simulink model "OcularMotorLabModel_2023_08_25_M22b"  (R2023a)
settings: Solver=FixedStepAuto  StartTime=tStart  StopTime=tFinal  FixedStep=0.001  RelTol=1e-3
undefined symbols (not defined in the file or in its folder): Asp, Asp1, Asp2, e0sp, gaussian, Gpc, GPos, Gsl, psi, Psp1, RotFbk, SatSp, sigbuilder_block, SomFbk, T1, T2, Tccanal, Tcn, Tcr, Tcsp, TCvs, tdm, tdsp1, tdsp2, tdsp3, tdv, Tsl, Tz, w
libraries: matrix_library x10, vrlib x8, simulink_extras x5, simulink x1
(part 1 of 2)
settings Model: Creator=raulr  LastModifiedBy=jom
settings DebuggingCC: UnconnectedInputMsg=warning  UnconnectedOutputMsg=warning  UnconnectedLineMsg=warning
settings ModelReferenceCC: EnableRefExpFcnMdlSchedulingChecks=on
settings RTWCC: DLArmComputeVersion=19.05

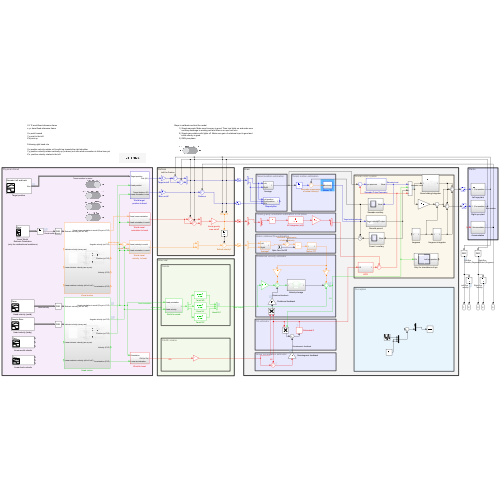
[thumbnail: Simulink's stored preview of the top-level diagram]
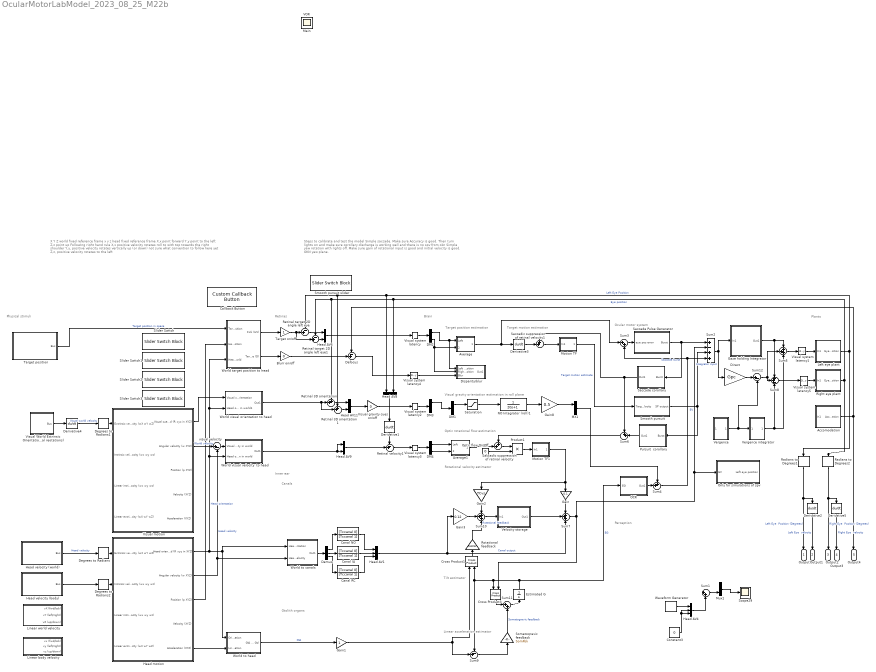
== system OcularMotorLabModel_2023_08_25_M22b ==
  note: Plants
  note: Steps to calibrate and test the model
      | Simple saccade. Make sure Accuracy is good. Then turn lights on and make sure corollary discharge is working well and there is no spv from okn
      | Simple yaw rotation with lights off. Make sure gain of rotational input is good and initial velocity is good.
      | OKN yaw plane.
  note: X Y Z world fixed reference frame
      | x y z head fixed reference frame
      |
      | X,x point forward
      | Y,y point to the left
      | Z,z point up
      |
      | Following right hand rule
      |
      | X,x positive velocity rotates roll to with top towards the right shoulder
      | Y,y, positive velocity rotates vertically up (or down) not sure what convention to follow here yet
      | Z,z, positive velocity rotates to the left
  note: Brain
  note: Ocular motor system
  note: Perception
  note: Optic rotational flow estimation
  note: Rotational velocity estimator
  note: Linear acceleration estimator
  note: Tilt estimator
  note: Retinas
  note: Otolith organs
  note: Canals
  note: Inner ear
  note: Physical stimuli
  note: Visual gravity orientation estimation in roll plane
  note: Target motion estimation
  note: Target position estimation
  Accomodation : Subsystem
  Average : Subsystem
  Average1 : Subsystem
  Blurr on/off : Gain  Gain=0
  Callback Button : CustomCallbackButton  Configuration="{\"components\":[{\"name\":\"BackgroundImageComponent\",\"settings\":{\"image\":{\"size\":[0,0],\"src\":\"default\",\"srcOrientation\":\"Right\"},\"position\":[0,0,1,1]}},{\"name\":\"ButtonStateComponent\",\"settings\":{\"buttonType\":\"momentary\",\"clickFcn\":\"%% Set parameters\\ntStart = 0;\\ntFinal = 60;\\n\\n\\n%% General\\ntdv = 0.050; % visual latency\\ntdm = 0.030; % Motor latency\\n\\n\\n%% plant\\nTz = 0.08;\\nT1 = 0.3;\\nT2 = 0.01; % 0.012\\nw = 200;\\npsi = 1.2;\\n\\n\\n%% Saccade system\\nGpc = 0.06;     % Gain of conjugate pulse\\nGsl = 0.165;    % Gain of slide\\nTsl = Tz;     % Tc slide\\nTcn = 20;       % Tc conjugate neural integrator\\nTcr = Tcn;       % Tc conjugate resettable integrator\\n\\nTep = 0.003;    % Tc motor error pole\\nDelC = 0.006;   % Saccade local feedback delay\\ne0 = 5;         \\nAL = 440;\\nAR = 440;\\nlL = 10;\\nLR = 10;\\n\\n%% Smooth pursuit\\ntdsp1 = 0.015;\\ntdsp2 = 0.035;\\ntdsp3 = 0.030;\\n\\nTcsp = 0.007;\\ne0sp = 4;\\nAsp1 = 10;\\nAsp2 = 5;\\nAsp = 1.1;\\nPsp1 = 0.95;\\nTcsp2 = 0.015;\\nSatSp = 90;\\n\\n%% Vestibular system\\nTccanal = 5;\\nTCvs = 11.5;\\nRotFbk = 0.38;\\nSomFbk = 0.65;\\n\\n%% Integrator\\nGPos = 0.02;\",\"onValue\":1,\"position\":[0,0,1,1],\"pressDelay\":\"500\",\"pressFcn\":\"\",\"repeatInterval\":\"0\",\"states\":[{\"horizontalAlignment\":\"center\",\"image\":{\"position\":[0,0,1,1],\"size\":[1,1],\"src\":\"default\",\"srcOrientation\":\"Right\"},\"label\":{\"color\":[0.01176470588,0.01176470588,0.01176470588,1],\"icon\":{\"size\":[0,0],\"src\":\"default\",\"srcOrientation\":\"Right\"},\"iconPlacement\":\"left\",\"opacity\":1,\"show\":true,\"text\":{\"content\":\"Click to initialize\",\"font\":\"Helvetica\",\"fontSize\":13.865820000000001}},\"labelOffset\":[0,0],\"verticalAlignment\":\"middle\"},{\"horizontalAlignment\":\"center\",\"image\":{\"position\":[0,0,1,1],\"size\":[1,1],\"src\":\"default\",\"srcOrientation\":\"Right\"},\"label\":{\"color\":[0.01176470588,0.01176470588,0.01176470588,1],\"icon\":{\"size\":[0,0],\"src\":\"default\",\"srcOrientation\":\"Right\"},\"iconPlacement\":\"left\",\"opacity\":1,\"show\":true,\"text\":{\"content\":\"Click to initialize\",\"font\":\"Helvetica\",\"fontSize\":13.865820000000001}},\"labelOffset\":[0,0],\"verticalAlignment\":\"middle\"},{\"horizontalAlignment\":\"center\",\"image\":{\"position\":[0,0,1,1],\"size\":[1,1],\"src\":\"default\",\"srcOrientation\":\"Right\"},\"label\":{\"color\":[0.01176470588,0.01176470588,0.01176470588,1],\"icon\":{\"size\":[0,0],\"src\":\"default\",\"srcOrientation\":\"Right\"},\"iconPlacement\":\"left\",\"opacity\":1,\"show\":true,\"text\":{\"content\":\"Click to initialize\",\"font\":\"Helvetica\",\"fontSize\":13.865820000000001}},\"labelOffset\":[0,0],\"verticalAlignment\":\"middle\"},{\"horizontalAlignment\":\"center\",\"image\":{\"position\":[0,0,1,1],\"size\":[1,1],\"src\":\"default\",\"srcOrientation\":\"Right\"},\"label\":{\"color\":[0.01176470588,0.01176470588,0.01176470588,1],\"icon\":{\"size\":[0,0],\"src\":\"default\",\"srcOrientation\":\"Right\"},\"iconPlacement\":\"left\",\"opacity\":1,\"show\":true,\"text\":{\"content\":\"Click to initialize\",\"font\":\"Helvetica\",\"fontSize\":13.865820000000001}},\"labelOffset\":[0,0],\"verticalAlignment\":\"middle\"}]}},{\"name\":\"ForegroundImageComponent\",\"settings\":{\"image\":{\"size\":[0,0],\"src\":\"default\",\"srcOrientation\":\"Right\"},\"isForeground\":1,\"position\":[0,0,1,1]}}],\"settings\":{\"BindingType\":\"standalone\",\"backgroundColor\":[244,244,244,1],\"backgroundOffset\":0.2,\"backgroundOpacity\":1,\"fixedAspectRatio\":\"off\",\"foregroundColor\":[0.01176470588,0.01176470588,0.01176470588,1],\"migratedFromLegacy\":true,\"useBackgroundColor\":true,\"variant\":\"callback\",\"version\":\"R2023a\"},\"type\":\"Button\"}"  CustomBackgroundColor="{\"color\":[0.9568627451,0.9568627451,0.9568627451],\"show\":true}"
  Canal IA : TransferFcn  Numerator=[Tccanal 0]  Denominator=[Tccanal 1]
  Canal NO : TransferFcn  Numerator=[Tccanal 0]  Denominator=[Tccanal 1]
  Canal RC : TransferFcn  Numerator=[Tccanal 0]  Denominator=[Tccanal 1]
  Constant3 : Constant  Value=0
  Cross Product1 : vrlib/Utilities/Cross Product
  Cross Product3 : vrlib/Utilities/Cross Product
  DM1 : Demux  Outputs=3
  DM2 : Demux  Outputs=2
  DM3 : Demux  Outputs=2
  DM4 : Demux  Outputs=2
  Defocus : Sum  Inputs=-+|
  Degrees to Radians : simulink_extras/Transformations/Degrees to Radians
  Degrees to Radians1 : simulink_extras/Transformations/Degrees to Radians
  Degrees to Radians2 : simulink_extras/Transformations/Degrees to Radians
  Demux : Demux  Outputs=3
  Derivative{1..5} (5 alike) : Derivative
  Direct : Gain  Gain=Gpc
  Disparity/blur : Subsystem
  Estimated G : Integrator  InitialCondition=[0 0 -1]'
  Gain : Gain  Gain=0.1
  Gain1 : Gain
  Gain2 : Gain  Gain=TCvs
  Gain3 : Gain  Gain=0.12
  Gain8 : Gain  Gain=0.5
  Gaze holding Integrator : Subsystem
  Head AV1 : Mux  Inputs=3
  Head AV{6,8..9,11} (4 alike) : Mux  Inputs=2
  Head AV4 : Mux  Inputs=3
  Head motion : Subsystem
  Head velocity (body) : Subsystem  Tag=STV Subsys  LoadFcn=sigbuilder_block('load');  StartFcn=sigbuilder_block('start');  StopFcn=sigbuilder_block('stop');  ClipboardFcn=sigbuilder_block('clipboard');  mask(Sigbuilder block){tuvar=[0:10]}
      mask help: Simulink:masks:SigbuilderBlock_MD
      mask init:
      | if ~strcmp(get_param(bdroot(gcbh),'SimulationStatus'),'stopped') tuvar = sigbuilder_block('maskInit'); end
      settings: CopyFcn=sigbuilder_block('copy');  DeleteFcn=sigbuilder_block('delete');  ModelCloseFcn=sigbuilder_block('modelClose');  PreSaveFcn=sigbuilder_block('preSave');  PauseFcn=sigbuilder_block('pause');  ContinueFcn=sigbuilder_block('continue');  NameChangeFcn=sigbuilder_block('namechange');  OpenFcn=sigbuilder_block('open',[5.4 5.4 1141.2 580.8 ]);  CloseFcn=sigbuilder_block('close');
      mask Display: plot(0, 0, 100, 100,[2, 2, 32, 32, 2], [68, 8, 8, 68, 68],[32, 2], [38, 38], [32, 19, 2],[53, 60, 44], [32, 17, 17, 2],[16, 16, 31, 31]);txt = getActiveGroup(gcbh);text(2, 100, txt,'verticalAlignment', 'top');
  Head velocity (world) : Subsystem  Tag=STV Subsys  LoadFcn=sigbuilder_block('load');  StartFcn=sigbuilder_block('start');  StopFcn=sigbuilder_block('stop');  ClipboardFcn=sigbuilder_block('clipboard');  mask(Sigbuilder block){tuvar=[0:10]}
      mask help: Simulink:masks:SigbuilderBlock_MD
      mask init:
      | if ~strcmp(get_param(bdroot(gcbh),'SimulationStatus'),'stopped') tuvar = sigbuilder_block('maskInit'); end
      settings: CopyFcn=sigbuilder_block('copy');  DeleteFcn=sigbuilder_block('delete');  ModelCloseFcn=sigbuilder_block('modelClose');  PreSaveFcn=sigbuilder_block('preSave');  PauseFcn=sigbuilder_block('pause');  ContinueFcn=sigbuilder_block('continue');  NameChangeFcn=sigbuilder_block('namechange');  OpenFcn=sigbuilder_block('open',[2616 248.4 1141.2 580.8 ]);  CloseFcn=sigbuilder_block('close');
      mask Display: plot(0, 0, 100, 100,[2, 2, 32, 32, 2], [68, 8, 8, 68, 68],[32, 2], [38, 38], [32, 19, 2],[53, 60, 44], [32, 17, 17, 2],[16, 16, 31, 31]);txt = getActiveGroup(gcbh);text(2, 100, txt,'verticalAlignment', 'top');
  Left eye plant : Subsystem
  Linear body velocity : Subsystem  Tag=STV Subsys  LoadFcn=sigbuilder_block('load');  StartFcn=sigbuilder_block('start');  StopFcn=sigbuilder_block('stop');  ClipboardFcn=sigbuilder_block('clipboard');  mask(Sigbuilder block){tuvar=[0:10]}
      mask help: Simulink:masks:SigbuilderBlock_MD
      mask init:
      | if ~strcmp(get_param(bdroot(gcbh),'SimulationStatus'),'stopped') tuvar = sigbuilder_block('maskInit'); end
      settings: CopyFcn=sigbuilder_block('copy');  DeleteFcn=sigbuilder_block('delete');  ModelCloseFcn=sigbuilder_block('modelClose');  PreSaveFcn=sigbuilder_block('preSave');  PauseFcn=sigbuilder_block('pause');  ContinueFcn=sigbuilder_block('continue');  NameChangeFcn=sigbuilder_block('namechange');  OpenFcn=sigbuilder_block('open',[352.5 317 1141 398 ]);  CloseFcn=sigbuilder_block('close');
      mask Display: plot(0, 0, 100, 100,[2, 2, 32, 32, 2], [68, 8, 8, 68, 68],[32, 2], [38, 38], [32, 19, 2],[53, 60, 44], [32, 17, 17, 2],[16, 16, 31, 31]);txt = getActiveGroup(gcbh);text(2, 100, txt,'verticalAlignment', 'top');
  Linear world velocity : Subsystem  Tag=STV Subsys  LoadFcn=sigbuilder_block('load');  StartFcn=sigbuilder_block('start');  StopFcn=sigbuilder_block('stop');  ClipboardFcn=sigbuilder_block('clipboard');  mask(Sigbuilder block){tuvar=[0:10]}
      mask help: Simulink:masks:SigbuilderBlock_MD
      mask init:
      | if ~strcmp(get_param(bdroot(gcbh),'SimulationStatus'),'stopped') tuvar = sigbuilder_block('maskInit'); end
      settings: CopyFcn=sigbuilder_block('copy');  DeleteFcn=sigbuilder_block('delete');  ModelCloseFcn=sigbuilder_block('modelClose');  PreSaveFcn=sigbuilder_block('preSave');  PauseFcn=sigbuilder_block('pause');  ContinueFcn=sigbuilder_block('continue');  NameChangeFcn=sigbuilder_block('namechange');  OpenFcn=sigbuilder_block('open',[448.5 188.5 1141 397.7 ]);  CloseFcn=sigbuilder_block('close');
      mask Display: plot(0, 0, 100, 100,[2, 2, 32, 32, 2], [68, 8, 8, 68, 68],[32, 2], [38, 38], [32, 19, 2],[53, 60, 44], [32, 17, 17, 2],[16, 16, 31, 31]);txt = getActiveGroup(gcbh);text(2, 100, txt,'verticalAlignment', 'top');
  MX1 : Mux  Inputs=3
  Motion TF : Subsystem
  Motion TF1 : Subsystem
  Mux1 : Mux  Inputs=2
  NO Integrator (roll)1 : TransferFcn  Denominator=[20 1]
  OCR : Subsystem
  Only for simulations of spv : Subsystem
  Optic flow On/Off : Constant  Value=0
  Product1 : Product
  Pursuit  corollary : Subsystem
  Radians to Degrees1 : simulink_extras/Transformations/Radians to Degrees
  Radians to Degrees2 : simulink_extras/Transformations/Radians to Degrees
  Retinal 3D orientation : Sum  Inputs=++|
  Retinal 3D orientation1 : Sum  Inputs=++|
  Retinal target 2D angle left eye : Sum  Inputs=-+|
  Retinal target 2D angle left eye1 : Sum  Inputs=-+|
  Retinal velocity1 : Sum  Inputs=-+|
  Right eye plant : Subsystem
  Rotational feedback : Gain  Gain=RotFbk
  Saccade Pulse Generator : Subsystem
  Saccade corollary : Subsystem
  Saccadic suppression of retinal velocity : Sum  Inputs=++|
  Saccadic suppression of retinal velocity1 : Sum  Inputs=++|
  Saturation : Saturate  UpperLimit=5*pi/180  LowerLimit=-5*pi/180
  Scope29 : Scope
  Slider Switch{,1..3} (4 alike) : SliderSwitchBlock
      settings: Values={{'Off', 'On'}, [0 1]}
  Smooth pursuit : Subsystem
  Smooth pursuit slider : SliderSwitchBlock
      settings: Values={{'Off', 'On'}, [0 1]}
  Somatogravic feedback : Gain  Gain=SomFbk
  Sum1 : Sum  Inputs=|++
  Sum10 : Sum  Inputs=+++
  Sum11 : Sum  Inputs=|++
  Sum12 : Sum  Inputs=|+-
  Sum2 : Sum  Inputs=+-++
  Sum3 : Sum  Inputs=|++
  Sum4 : Sum  Inputs=++|
  Sum5 : Sum  Inputs=+++
  Sum6 : Sum  Inputs=++|
  Sum7 : Sum  Inputs=+++
  Sum8 : Sum  Inputs=++-
  Sum9 : Sum  Inputs=-+|
  Target on/off : Gain
  Target position : Subsystem  Tag=STV Subsys  LoadFcn=sigbuilder_block('load');  StartFcn=sigbuilder_block('start');  StopFcn=sigbuilder_block('stop');  ClipboardFcn=sigbuilder_block('clipboard');  mask(Sigbuilder block){tuvar=[0:10]}
      mask help: Simulink:masks:SigbuilderBlock_MD
      mask init:
      | if ~strcmp(get_param(bdroot(gcbh),'SimulationStatus'),'stopped') tuvar = sigbuilder_block('maskInit'); end
      settings: CopyFcn=sigbuilder_block('copy');  DeleteFcn=sigbuilder_block('delete');  ModelCloseFcn=sigbuilder_block('modelClose');  PreSaveFcn=sigbuilder_block('preSave');  PauseFcn=sigbuilder_block('pause');  ContinueFcn=sigbuilder_block('continue');  NameChangeFcn=sigbuilder_block('namechange');  OpenFcn=sigbuilder_block('open',[2766.6 334.8 1141.2 502.8 ]);  CloseFcn=sigbuilder_block('close');
      mask Display: plot(0, 0, 100, 100,[2, 2, 32, 32, 2], [68, 8, 8, 68, 68],[32, 2], [38, 38], [32, 19, 2],[53, 60, 44], [32, 17, 17, 2],[16, 16, 31, 31]);txt = getActiveGroup(gcbh);text(2, 100, txt,'verticalAlignment', 'top');
  Velocity storage : Subsystem
  Vergence : Subsystem
  Vergence integrator : Subsystem
  Visual World Extrinsic Orientation (only for unidirectional reotations) : Subsystem  Tag=STV Subsys  LoadFcn=sigbuilder_block('load');  StartFcn=sigbuilder_block('start');  StopFcn=sigbuilder_block('stop');  ClipboardFcn=sigbuilder_block('clipboard');  mask(Sigbuilder block){tuvar=[0:10]}
      mask help: Simulink:masks:SigbuilderBlock_MD
      mask init:
      | if ~strcmp(get_param(bdroot(gcbh),'SimulationStatus'),'stopped') tuvar = sigbuilder_block('maskInit'); end
      settings: CopyFcn=sigbuilder_block('copy');  DeleteFcn=sigbuilder_block('delete');  ModelCloseFcn=sigbuilder_block('modelClose');  PreSaveFcn=sigbuilder_block('preSave');  PauseFcn=sigbuilder_block('pause');  ContinueFcn=sigbuilder_block('continue');  NameChangeFcn=sigbuilder_block('namechange');  OpenFcn=sigbuilder_block('open',[389.4 19.2 1909.2 907.8 ]);  CloseFcn=sigbuilder_block('close');
      mask Display: plot(0, 0, 100, 100,[2, 2, 32, 32, 2], [68, 8, 8, 68, 68],[32, 2], [38, 38], [32, 19, 2],[53, 60, 44], [32, 17, 17, 2],[16, 16, 31, 31]);txt = getActiveGroup(gcbh);text(2, 100, txt,'verticalAlignment', 'top');
  Visual gravity cues on/off : Gain  Gain=0
  Visual motion : Subsystem
  Visual system latency{,2..4} (4 alike) : TransportDelay  DelayTime=tdv
  Visual system latency1 : TransportDelay  DelayTime=tdm
  Visual system latency5 : TransportDelay  DelayTime=tdm
  Waveform Generator : simulink/Sources/Waveform Generator  OutMin=[]  OutMax=[]  OutDataTypeStr=double  SelectedSignal=1  Signals=gaussian(0,0.1,1)  BlockNames=MultiportSwitch_125da93d47db44d  SampleTime=0.1
  World target position to head : Subsystem
  World to canals : Subsystem
  World to head : Subsystem
  World visual orientation to head : Subsystem
  World visual velocity  to head : Subsystem
  visual velocity : Sum  Inputs=|+-
  Output : Outport
  Output1 : Outport  Port=2
  Output2 : Outport  Port=3
  Output3 : Outport  Port=4
  Output4 : Outport  Port=5
  Main : Scope
  VOR : Scope
  wires:
  Sum7/1 -> Only for simulations of spv/1(EV), Sum2/2, Cross Product3/2  "EV"
  Sum9/1 -> Somatogravic feedback/1
  Cross Product3/1 -> Sum11/1
  Estimated G/1 -> Cross Product3/1, Sum9/1, Cross Product1/2, OCR/1(EG)  "EG"
  Cross Product1/1 -> Rotational feedback/1
  Demux/1 -> Canal NO/1
  Demux/2 -> Canal IA/1
  Canal IA/1 -> Head AV1/2
  Canal NO/1 -> Head AV1/1
  Canal RC/1 -> Head AV1/3
  Demux/3 -> Canal RC/1
  Head AV1/1 -> Gain3/1, Sum7/3  "Canal output"
  Head velocity (world)/1(Bus) -> Degrees to Radians/1  "Head velocity"
  Sum11/1 -> Estimated G/1
  Rotational feedback/1 -> Sum10/3  "Rotational feedback"
  Somatogravic feedback/1 -> Sum11/2  "Somatogravic feedback"
  Gaze holding Integrator/1(Out1) -> Sum5/1, Sum8/1
  Gain1/1 -> Cross Product1/1, Sum9/2
  Gain3/1 -> Sum10/2
  Motion TF1/1(Out1) -> Gain/1, Gain2/1
  Gain/1 -> Sum7/1
  Radians to Degrees1/1 -> Derivative2/1, Output/1  "Left Eye  Position (Degrees)"
  NO Integrator (roll)1/1 -> Gain8/1
  MX1/1 -> Sum4/1
  Derivative4/1 -> Degrees to Radians1/1  "Visual world velocity"
  Sum1/1 -> Mux1/2
  Mux1/1 -> Scope29/1
  Constant3/1 -> Head AV4/2, Head AV4/3
  Waveform Generator/1 -> Head AV4/1
  Head AV4/1 -> Sum1/2
  Saccade Pulse Generator/1(Burst) -> Saccade corollary/1(Burst), Sum2/1  "Saccade burst"
  Sum2/1 -> Direct/1, Gaze holding Integrator/1(In1)  "Integrator input"
  Product1/1 -> Motion TF1/1(In1)
  Saccadic suppression of retinal velocity/1 -> Product1/1
  Sum4/1 -> Sum3/2, Sum2/4
  Head velocity (body)/1(Bus) -> Degrees to Radians2/1
  Degrees to Radians2/1 -> Head motion/2(Intrinsic velocity (wx wy wz))
  Degrees to Radians/1 -> Head motion/1(Extrinsic velocity (wX wY wZ))
  Head motion/1(Head orientation in world (R xyz in XYZ)) -> World to canals/1(Head orientation), World to head/1(Orientation), World visual velocity  to head/2(Head orientation in world), World target position to head/3(Head orientation in world), World visual orientation to head/2(Head orientation in world1)  "Head orientation"
  Head motion/5(Acceleration (XYZ)) -> World to head/2(Linear acceleration)
  Head motion/2(Angular velocity (w XYZ)) -> visual velocity/2, World to canals/2(Head velocity)  "Head velocity"
  Degrees to Radians1/1 -> Visual motion/1(Extrinsic velocity (wX wY wZ))
  visual velocity/1 -> World visual velocity  to head/1(Visual velocity in world)
  Target position/1(Bus) -> World target position to head/1(Target position)  "Target position in space"
  Head motion/3(Position (p XYZ)) -> World target position to head/2(Head position)
  Visual motion/1(Visual cues orientation in world (R xyz in XYZ)) -> World visual orientation to head/1(Visual cues orientation)
  Visual motion/2(Angular velocity (w XYZ)) -> visual velocity/1  "World velocity"
  World visual velocity  to head/1(Out1) -> Head AV9/2, Head AV9/1
  World to canals/1(Out1) -> Demux/1
  World target position to head/1(Fick (HV)) -> Target on/off/1
  World to head/1(GIA (in Gs)) -> Gain1/1  "GIA"
  Sum3/1 -> Saccade Pulse Generator/1(eye pos error)
  OCR/1(Out1) -> Sum4/2
  Saturation/1 -> NO Integrator (roll)1/1
  Optic flow On/Off/1 -> Product1/2
  DM1/1 -> Saturation/1
  Gain8/1 -> MX1/1
  Average/1(Out1) -> Sum3/1, Derivative3/1
  Motion TF/1(Target velocity) -> Smooth pursuit/1(Target velocity)  "Target motion estimate"
  DM2/1 -> Disparity/blur/1(Left position), Average/1(Left)
  DM3/1 -> DM1/1
  Retinal velocity1/1 -> Visual system latency3/1
  Gain2/1 -> Sum10/1
  Derivative1/1 -> Retinal velocity1/1
  Visual system latency3/1 -> DM4/1
  Saccade corollary/1(Out1) -> Saccadic suppression of retinal velocity1/1, Sum6/1
  Smooth pursuit/1(SP output) -> Sum2/3, Pursuit  corollary/1(Burst)
  World target position to head/2(Target distance (D)) -> Blurr on/off/1
  Defocus/1 -> Visual system latency4/1
  Head AV6/1 -> Visual system latency/1
  DM2/2 -> Average/2(Right), Disparity/blur/2(Right position)
  Visual system latency4/1 -> Disparity/blur/3(Blur)
  Average1/1(Out1) -> Saccadic suppression of retinal velocity/2
  DM4/2 -> Average1/2(Right)
  Visual system latency/1 -> DM2/1
  Visual system latency2/1 -> DM3/1
  Head AV8/1 -> Derivative1/1
  DM4/1 -> Average1/1(Left)
  Head AV9/1 -> Retinal velocity1/2
  Target on/off/1 -> Retinal target 2D angle left eye1/2, Retinal target 2D angle left eye/2
  World visual orientation to head/1(Out1) -> Retinal 3D orientation/2, Retinal 3D orientation1/2
  Retinal target 2D angle left eye/1 -> Head AV6/1
  Retinal target 2D angle left eye1/1 -> Head AV6/2
  Derivative3/1 -> Saccadic suppression of retinal velocity1/2
  Saccadic suppression of retinal velocity1/1 -> Motion TF/1(In1)
  Sum6/1 -> Saccadic suppression of retinal velocity/1
  Pursuit  corollary/1(Out1) -> Sum6/2
  Right eye plant/1(Eye position) -> Radians to Degrees2/1, Head AV8/2, Retinal 3D orientation/1, Retinal target 2D angle left eye1/1  "Eye position"
  Sum8/1 -> Visual system latency5/1
  Accomodation/1(Accomodation) -> Output4/1, Defocus/1
  ? -> Accomodation/1(In1)
  Sum5/1 -> Visual system latency1/1
  Left eye plant/1(Eye position) -> Radians to Degrees1/1, Retinal target 2D angle left eye/1, Retinal 3D orientation1/1, Head AV8/1  "Left Eye Position"
  Blurr on/off/1 -> Defocus/2
  Retinal 3D orientation1/1 -> Head AV11/2
  Retinal 3D orientation/1 -> Head AV11/1
  Head AV11/1 -> Visual gravity cues on/off/1
  Vergence/1(Out1) -> Vergence integrator/1(In1), Sum12/2
  Sum12/1 -> Sum8/2, Sum5/2
  Direct/1 -> Sum12/1
  Vergence integrator/1(Out1) -> Sum8/3, Sum5/3
  Visual system latency1/1 -> Left eye plant/1(In1)
  Visual system latency5/1 -> Right eye plant/1(In1)
  Sum10/1 -> Velocity storage/1(In1)
  Velocity storage/1(Out1) -> Sum7/2
  Visual gravity cues on/off/1 -> Visual system latency2/1
  Derivative2/1 -> Output1/1  "Left Eye  velocity"
  Derivative5/1 -> Output3/1  "Right Eye  velocity"
  Radians to Degrees2/1 -> Derivative5/1, Output2/1  "Right Eye  Position (Degrees)"
  Visual World Extrinsic Orientation (only for unidirectional reotations)/1(Bus) -> Derivative4/1

== system OcularMotorLabModel_2023_08_25_M22b/Accomodation ==
  In1 : Inport
  Accomodation : Outport

== system OcularMotorLabModel_2023_08_25_M22b/Average ==
  Left : Inport
  Right : Inport  Port=2
  Constant : Constant  Value=2
  Divide : Product  Inputs=*/
  Sum : Sum  Inputs=|++
  Out1 : Outport
  wires:
  Divide/1 -> Out1/1
  Sum/1 -> Divide/1
  Left/1 -> Sum/1
  Constant/1 -> Divide/2
  Right/1 -> Sum/2

== system OcularMotorLabModel_2023_08_25_M22b/Average1 ==
  Left : Inport
  Right : Inport  Port=2
  Constant : Constant  Value=2
  Divide : Product  Inputs=*/
  Sum : Sum  Inputs=|++
  Out1 : Outport
  wires:
  Divide/1 -> Out1/1
  Sum/1 -> Divide/1
  Left/1 -> Sum/1
  Constant/1 -> Divide/2
  Right/1 -> Sum/2

== system OcularMotorLabModel_2023_08_25_M22b/Disparity//blur ==
  Left position : Inport
  Right position : Inport  Port=2
  Blur : Inport  Port=3
  Out1 : Outport

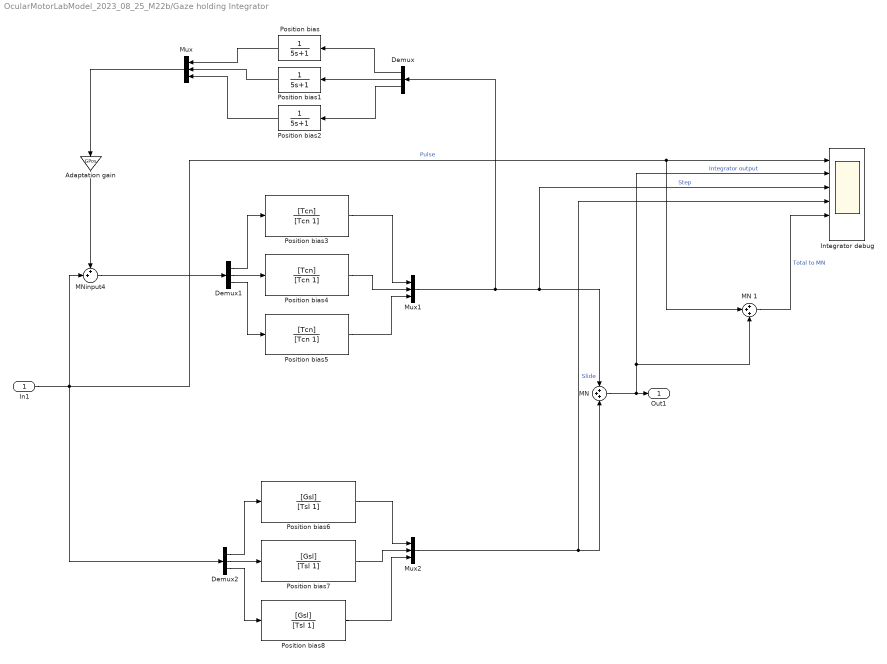
== system OcularMotorLabModel_2023_08_25_M22b/Gaze holding Integrator ==
  In1 : Inport
  Adaptation gain : Gain  Gain=GPos
  Demux : Demux  Outputs=3
  Demux1 : Demux  Outputs=3
  Demux2 : Demux  Outputs=3
  Integrator debug : Scope  NumInputPorts=6
  "MN " : Sum  Inputs=+++  InputSameDT=on  SaturateOnIntegerOverflow=on  OutDataTypeStr=Inherit: Same as first input
  MN 1 : Sum  Inputs=+++  InputSameDT=on  SaturateOnIntegerOverflow=on  OutDataTypeStr=Inherit: Same as first input
  MNinput4 : Sum  Inputs=++|  InputSameDT=on  SaturateOnIntegerOverflow=on  OutDataTypeStr=Inherit: Same as first input
  Mux : Mux  Inputs=3
  Mux1 : Mux  Inputs=3
  Mux2 : Mux  Inputs=3
  Position bias : TransferFcn  Numerator=1  Denominator=[5 1]
  Position bias1 : TransferFcn  Numerator=1  Denominator=[5 1]
  Position bias2 : TransferFcn  Numerator=1  Denominator=[5 1]
  Position bias3 : TransferFcn  Numerator=[Tcn]  Denominator=[Tcn 1]
  Position bias4 : TransferFcn  Numerator=[Tcn]  Denominator=[Tcn 1]
  Position bias5 : TransferFcn  Numerator=[Tcn]  Denominator=[Tcn 1]
  Position bias6 : TransferFcn  Numerator=[Gsl]  Denominator=[Tsl 1]
  Position bias7 : TransferFcn  Numerator=[Gsl]  Denominator=[Tsl 1]
  Position bias8 : TransferFcn  Numerator=[Gsl]  Denominator=[Tsl 1]
  Out1 : Outport
  wires:
  Mux/1 -> Adaptation gain/1
  Demux/1 -> Position bias/1
  Demux/2 -> Position bias1/1
  Demux/3 -> Position bias2/1
  Position bias1/1 -> Mux/2
  Position bias/1 -> Mux/1
  Position bias2/1 -> Mux/3
  MNinput4/1 -> Demux1/1
  Position bias4/1 -> Mux1/2
  Demux1/3 -> Position bias5/1
  Mux1/1 -> Demux/1, Integrator debug/3, "MN "/1  "Step"
  Position bias5/1 -> Mux1/3
  Position bias3/1 -> Mux1/1
  Demux1/2 -> Position bias4/1
  Demux1/1 -> Position bias3/1
  Position bias7/1 -> Mux2/2
  In1/1 -> MN 1/2, Integrator debug/1, MNinput4/2, Demux2/1  "Pulse"
  Demux2/1 -> Position bias6/1
  Position bias6/1 -> Mux2/1
  Demux2/3 -> Position bias8/1
  Position bias8/1 -> Mux2/3
  Demux2/2 -> Position bias7/1
  Mux2/1 -> "MN "/3, Integrator debug/4  "Slide"
  "MN "/1 -> MN 1/3, Integrator debug/2, Out1/1  "Integrator output"
  Adaptation gain/1 -> MNinput4/1
  MN 1/1 -> Integrator debug/5  "Total to MN"

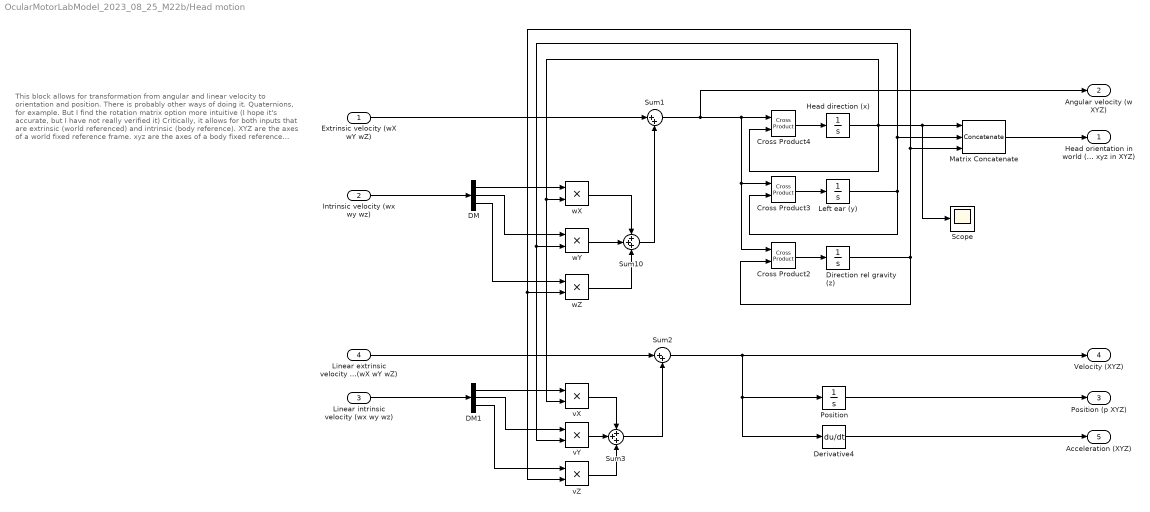
== system OcularMotorLabModel_2023_08_25_M22b/Head motion ==
  note: This block allows for transformation from angular and linear velocity to orientation and position. There is probably other ways of doing it. Quaternions, for example. But I find the rotation matrix option more intuitive (I hope it's accurate, but I have not really verified it)
      |
      | Critically, it allows for both inputs that are extrinsic (world referenced) and intrinsic (body reference).
      |
      | XYZ are the axes of a world fixed reference frame.
      | xyz are the axes of a body fixed reference frame
      |
      | For the extrinsic angular velocities, they need to be integrated after a cross product with each of the xyz axis, that way they provide the rotation of such axis within the XYZ world fixed reference frame.
      |
      | For the intrinsic angular velocities, they simply multiply each of the intrisic axis and get added to the extrinsic velocities.
      |
      | A similar approach is followed for the linear velocities but without the cross products are linear velocities can be simply integrated by components.
  Extrinsic velocity (wX wY wZ) : Inport
  Intrinsic velocity (wx wy wz) : Inport  Port=2
  Linear intrinsic velocity (wx wy wz) : Inport  Port=3
  Linear extrinsic velocity (wX wY wZ) : Inport  Port=4
  Cross Product2 : vrlib/Utilities/Cross Product
  Cross Product3 : vrlib/Utilities/Cross Product
  Cross Product4 : vrlib/Utilities/Cross Product
  DM : Demux  Outputs=3
  DM1 : Demux  Outputs=3
  Derivative4 : Derivative
  Direction rel gravity (z) : Integrator  InitialCondition=[0 0 1]
  Head direction (x) : Integrator  InitialCondition=[1 0 0]
  Left ear (y) : Integrator  InitialCondition=[0 1 0]
  Matrix Concatenate : Concatenate  NumInputs=3  Mode=Multidimensional array  ConcatenateDimension=2
  Position : Integrator  InitialCondition=[0 0 0]
  Scope : Scope
  Sum1 : Sum  Inputs=|++
  Sum10 : Sum  Inputs=+++
  Sum2 : Sum  Inputs=|++
  Sum3 : Sum  Inputs=+++
  vX : Product
  vY : Product
  vZ : Product
  wX : Product
  wY : Product
  wZ : Product
  Head orientation in world (R xyz in XYZ) : Outport
  Angular velocity (w XYZ) : Outport  Port=2
  Position (p XYZ) : Outport  Port=3
  Velocity (XYZ) : Outport  Port=4
  Acceleration (XYZ) : Outport  Port=5
  wires:
  Head direction (x)/1 -> Scope/1, Matrix Concatenate/1, Cross Product4/2, wX/2, vX/2
  Cross Product4/1 -> Head direction (x)/1
  Direction rel gravity (z)/1 -> Matrix Concatenate/3, wZ/2, vZ/2, Cross Product2/2
  Cross Product2/1 -> Direction rel gravity (z)/1
  Left ear (y)/1 -> Matrix Concatenate/2, vY/2, wY/2, Cross Product3/2
  Sum1/1 -> Cross Product2/1, Cross Product3/1, Cross Product4/1, Angular velocity (w XYZ)/1
  Cross Product3/1 -> Left ear (y)/1
  DM/1 -> wX/1
  DM/2 -> wY/1
  DM/3 -> wZ/1
  wX/1 -> Sum10/1
  wY/1 -> Sum10/2
  wZ/1 -> Sum10/3
  Sum10/1 -> Sum1/2
  Position/1 -> Position (p XYZ)/1
  vY/1 -> Sum3/2
  DM1/2 -> vY/1
  vZ/1 -> Sum3/3
  DM1/3 -> vZ/1
  DM1/1 -> vX/1
  vX/1 -> Sum3/1
  Sum3/1 -> Sum2/2
  Matrix Concatenate/1 -> Head orientation in world (R xyz in XYZ)/1
  Sum2/1 -> Position/1, Derivative4/1, Velocity (XYZ)/1
  Derivative4/1 -> Acceleration (XYZ)/1
  Extrinsic velocity (wX wY wZ)/1 -> Sum1/1
  Intrinsic velocity (wx wy wz)/1 -> DM/1
  Linear extrinsic velocity (wX wY wZ)/1 -> Sum2/1
  Linear intrinsic velocity (wx wy wz)/1 -> DM1/1

== system OcularMotorLabModel_2023_08_25_M22b/Head velocity (body) ==
  Bus Creator : BusCreator  Tag=Bus Creator  Inputs=3
  FromWs : FromWorkspace  Tag=STV FromWs  VariableName=tuvar
      SigBuilderData=|
      | common.afterFinalStr = 'Extrapolate'
      | common.sampleTime = 0
      | dataSet(1).timeRange = [0 40]
      | dataSet(1).name = 'Zeros'
      | dataSet(2).timeRange = [0 60]
      | dataSet(2).name = 'Sample Sims'
      | sbobj.Groups(1).Name = 'Zeros'
      | sbobj.Groups(1).Signals(1).Name = 'nasooccipital'
      | sbobj.Groups(1).Signals(1).XData = [0 5 6 15 40]
      | sbobj.Groups(1).Signals(1).YData = [0 0 0 0 0]
      | sbobj.Groups(1).Signals(2).Name = 'interaural'
      | sbobj.Groups(1).Signals(2).XData = [0 5 6 40]
      | sbobj.Groups(1).Signals(2).YData = [0 0 0 0]
      | sbobj.Groups(1).Signals(3).Name = 'rostrocaudal'
      | sbobj.Groups(1).Signals(3).XData = [0 5 15 40]
      | sbobj.Groups(1).Signals(3).YData = [0 0 0 0]
      | sbobj.Groups(1).TimeRange = [0 40]
      | sbobj.Groups(2).Name = 'Sample Sims'
      | sbobj.Groups(2).Signals(1).Name = 'nasooccipital'
      | sbobj.Groups(2).Signals(1).XData = [0 5 60]
      | sbobj.Groups(2).Signals(1).YData = [0 0 0]
      | sbobj.Groups(2).Signals(2).Name = 'interaural'
      | sbobj.Groups(2).Signals(2).XData = [0 5 35 60]
      | sbobj.Groups(2).Signals(2).YData = [0 0 0 0]
      | sbobj.Groups(2).Signals(3).Name = 'rostrocaudal'
      | sbobj.Groups(2).Signals(3).XData = [0 5 35 60]
      | sbobj.Groups(2).Signals(3).YData = [0 0 0 0]
      | sbobj.Groups(2).TimeRange = [0 60]
  Subsystem : Subsystem
  Bus : Outport
  wires:
  FromWs/1 -> Subsystem/1(In1)
  Subsystem/1(nasooccipital) -> Bus Creator/1  "nasooccipital"
  Subsystem/2(interaural) -> Bus Creator/2  "interaural"
  Subsystem/3(rostrocaudal) -> Bus Creator/3  "rostrocaudal"
  Bus Creator/1 -> Bus/1

== system OcularMotorLabModel_2023_08_25_M22b/Head velocity (world) ==
  Bus Creator : BusCreator  Tag=Bus Creator  Inputs=3
  FromWs : FromWorkspace  Tag=STV FromWs  VariableName=tuvar
      SigBuilderData=|
      | common.afterFinalStr = 'Extrapolate'
      | common.sampleTime = 0
      | dataSet(1).timeRange = [0 40]
      | dataSet(1).name = 'Zeros'
      | dataSet(2).timeRange = [0 60]
      | dataSet(2).name = 'Sample Sims'
      | dataSet(3).timeRange = [0 40]
      | dataSet(3).name = 'Zeros1'
      | sbobj.Groups(1).Name = 'Zeros'
      | sbobj.Groups(1).Signals(1).Name = 'nasooccipital'
      | sbobj.Groups(1).Signals(1).XData = [0 5 6 15 40]
      | sbobj.Groups(1).Signals(1).YData = [0 0 0 0 0]
      | sbobj.Groups(1).Signals(2).Name = 'interaural'
      | sbobj.Groups(1).Signals(2).XData = [0 5 6 40]
      | sbobj.Groups(1).Signals(2).YData = [0 0 0 0]
      | sbobj.Groups(1).Signals(3).Name = 'rostrocaudal'
      | sbobj.Groups(1).Signals(3).XData = [0 5 15 40]
      | sbobj.Groups(1).Signals(3).YData = [0 0 0 0]
      | sbobj.Groups(1).TimeRange = [0 40]
      | sbobj.Groups(2).Name = 'Sample Sims'
      | sbobj.Groups(2).Signals(1).Name = 'nasooccipital'
      | sbobj.Groups(2).Signals(1).XData = [0 5 60]
      | sbobj.Groups(2).Signals(1).YData = [0 0 0]
      | sbobj.Groups(2).Signals(2).Name = 'interaural'
      | sbobj.Groups(2).Signals(2).XData = [0 5 35 60]
      | sbobj.Groups(2).Signals(2).YData = [0 0 0 0]
      | sbobj.Groups(2).Signals(3).Name = 'rostrocaudal'
      | sbobj.Groups(2).Signals(3).XData = [0 5 35 60]
      | sbobj.Groups(2).Signals(3).YData = [0 0 0 0]
      | sbobj.Groups(2).TimeRange = [0 60]
      | sbobj.Groups(3).Name = 'Zeros1'
      | sbobj.Groups(3).Signals(1).Name = 'nasooccipital'
      | sbobj.Groups(3).Signals(1).XData = [0 5 6 15 40]
      | sbobj.Groups(3).Signals(1).YData = [0 0 0 0 0]
      | sbobj.Groups(3).Signals(2).Name = 'interaural'
      | sbobj.Groups(3).Signals(2).XData = [0 5 6 40]
      | sbobj.Groups(3).Signals(2).YData = [0 0 0 0]
      | sbobj.Groups(3).Signals(3).Name = 'rostrocaudal'
      | sbobj.Groups(3).Signals(3).XData = [0 5 15 40]
      | sbobj.Groups(3).Signals(3).YData = [0 0 0 0]
      | sbobj.Groups(3).TimeRange = [0 40]
  Subsystem : Subsystem
  Bus : Outport
  wires:
  FromWs/1 -> Subsystem/1(In1)
  Subsystem/1(nasooccipital) -> Bus Creator/1  "nasooccipital"
  Subsystem/2(interaural) -> Bus Creator/2  "interaural"
  Subsystem/3(rostrocaudal) -> Bus Creator/3  "rostrocaudal"
  Bus Creator/1 -> Bus/1

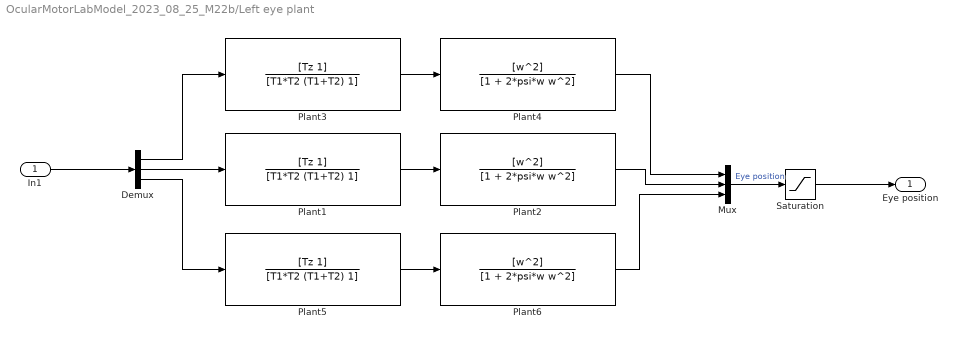
== system OcularMotorLabModel_2023_08_25_M22b/Left eye plant ==
  In1 : Inport
  Demux : Demux  Outputs=3
  Mux : Mux  Inputs=3
  Plant1 : TransferFcn  Numerator=[Tz 1]  Denominator=[T1*T2 (T1+T2) 1]
  Plant2 : TransferFcn  Numerator=[w^2]  Denominator=[1 + 2*psi*w w^2]
  Plant3 : TransferFcn  Numerator=[Tz 1]  Denominator=[T1*T2 (T1+T2) 1]
  Plant4 : TransferFcn  Numerator=[w^2]  Denominator=[1 + 2*psi*w w^2]
  Plant5 : TransferFcn  Numerator=[Tz 1]  Denominator=[T1*T2 (T1+T2) 1]
  Plant6 : TransferFcn  Numerator=[w^2]  Denominator=[1 + 2*psi*w w^2]
  Saturation : Saturate  UpperLimit=50*pi/180  LowerLimit=-50*pi/180
  Eye position : Outport
  wires:
  In1/1 -> Demux/1
  Mux/1 -> Saturation/1  "Eye position"
  Plant4/1 -> Mux/1
  Plant2/1 -> Mux/2
  Plant6/1 -> Mux/3
  Demux/1 -> Plant3/1
  Demux/2 -> Plant1/1
  Demux/3 -> Plant5/1
  Saturation/1 -> Eye position/1
  Plant3/1 -> Plant4/1
  Plant1/1 -> Plant2/1
  Plant5/1 -> Plant6/1

== system OcularMotorLabModel_2023_08_25_M22b/Linear body velocity ==
  Demux : Demux  Tag=STV Demux  Outputs=3
      settings: DisplayOption=none
  FromWs : FromWorkspace  Tag=STV FromWs  VariableName=tuvar
      SigBuilderData=|
      | common.afterFinalStr = 'Extrapolate'
      | common.sampleTime = 0
      | dataSet.timeRange = [0 60]
      | dataSet.name = 'Zero'
      | sbobj.Groups.Name = 'Zero'
      | sbobj.Groups.Signals(1).Name = 'vx (fwd/bck)'
      | sbobj.Groups.Signals(1).XData = [0 60]
      | sbobj.Groups.Signals(1).YData = [0 0]
      | sbobj.Groups.Signals(2).Name = 'vy (left/right)'
      | sbobj.Groups.Signals(2).XData = [0 10 12 20 22 60]
      | sbobj.Groups.Signals(2).YData = [0 0 0 0 0 0]
      | sbobj.Groups.Signals(3).Name = 'vz (up/down)'
      | sbobj.Groups.Signals(3).XData = [0 60]
      | sbobj.Groups.Signals(3).YData = [0 0]
      | sbobj.Groups.TimeRange = [0 60]
  Subsystem : Subsystem
  vx (fwd/bck) : Outport  Tag=STV Outport
  vy (left/right) : Outport  Tag=STV Outport  Port=2
  vz (up/down) : Outport  Tag=STV Outport  Port=3
  wires:
  FromWs/1 -> Demux/1
  Demux/1 -> vx (fwd/bck)/1
  Demux/2 -> vy (left/right)/1
  Demux/3 -> vz (up/down)/1

== system OcularMotorLabModel_2023_08_25_M22b/Linear world velocity ==
  Demux : Demux  Tag=STV Demux  Outputs=3
      settings: DisplayOption=none
  FromWs : FromWorkspace  Tag=STV FromWs  VariableName=tuvar
      SigBuilderData=|
      | common.afterFinalStr = 'Extrapolate'
      | common.sampleTime = 0
      | dataSet.timeRange = [0 60]
      | dataSet.name = 'Zero'
      | sbobj.Groups.Name = 'Zero'
      | sbobj.Groups.Signals(1).Name = 'vX (fwd/bck)'
      | sbobj.Groups.Signals(1).XData = [0 60]
      | sbobj.Groups.Signals(1).YData = [0 0]
      | sbobj.Groups.Signals(2).Name = 'vY (left/right)'
      | sbobj.Groups.Signals(2).XData = [0 10 12 20 22 60]
      | sbobj.Groups.Signals(2).YData = [0 0 0 0 0 0]
      | sbobj.Groups.Signals(3).Name = 'vZ (up/down)'
      | sbobj.Groups.Signals(3).XData = [0 60]
      | sbobj.Groups.Signals(3).YData = [0 0]
      | sbobj.Groups.TimeRange = [0 60]
  Subsystem : Subsystem
  vX (fwd/bck) : Outport  Tag=STV Outport
  vY (left/right) : Outport  Tag=STV Outport  Port=2
  vZ (up/down) : Outport  Tag=STV Outport  Port=3
  wires:
  FromWs/1 -> Demux/1
  Demux/1 -> vX (fwd/bck)/1
  Demux/2 -> vY (left/right)/1
  Demux/3 -> vZ (up/down)/1

== system OcularMotorLabModel_2023_08_25_M22b/Motion TF ==
  note: Symmetric Non linear function that grows linearly up to 50 deg/s (gain of 1) then decreases linearly up to 100 deg/s (gain from 1 gradually to 0) and it's zero after 100 deg/s
      |
      | Aims to simulate how we cannot track visual motion when it is too fast
  In1 : Inport
  Gain5 : Gain  Gain=2
  Saturation2 : Saturate  UpperLimit=50*pi/180  LowerLimit=-50*pi/180
  Saturation3 : Saturate  UpperLimit=100*pi/180  LowerLimit=-100*pi/180
  Sum8 : Sum  Inputs=+|-
  Target velocity : Outport
  wires:
  In1/1 -> Saturation3/1, Saturation2/1
  Saturation2/1 -> Gain5/1
  Saturation3/1 -> Sum8/2
  Gain5/1 -> Sum8/1
  Sum8/1 -> Target velocity/1

== system OcularMotorLabModel_2023_08_25_M22b/Motion TF1 ==
  note: Symmetric Non linear function that grows linearly up to 50 deg/s (gain of 1) then decreases linearly up to 100 deg/s (gain from 1 gradually to 0) and it's zero after 100 deg/s
      |
      | Aims to simulate how we cannot track visual motion when it is too fast
  In1 : Inport
  Gain4 : Gain  Gain=-1
  Gain5 : Gain  Gain=2
  Saturation2 : Saturate  UpperLimit=50*pi/180  LowerLimit=-50*pi/180
  Saturation3 : Saturate  UpperLimit=100*pi/180  LowerLimit=-100*pi/180
  Scope : Scope  NumInputPorts=3
  Sum8 : Sum  Inputs=+|-
  Out1 : Outport
  wires:
  In1/1 -> Gain4/1
  Saturation2/1 -> Gain5/1
  Saturation3/1 -> Scope/2, Sum8/2
  Gain5/1 -> Scope/1, Sum8/1
  Sum8/1 -> Scope/3, Out1/1
  Gain4/1 -> Saturation3/1, Saturation2/1

== system OcularMotorLabModel_2023_08_25_M22b/OCR ==
  EG : Inport
  Asin : Trigonometry  Operator=asin
  DM : Demux  Outputs=3
  Gain7 : Gain  Gain=-0.1
  MX : Mux  Inputs=3
  Out1 : Outport
  wires:
  Asin/1 -> Gain7/1
  Gain7/1 -> MX/1
  EG/1 -> DM/1
  DM/2 -> Asin/1
  MX/1 -> Out1/1

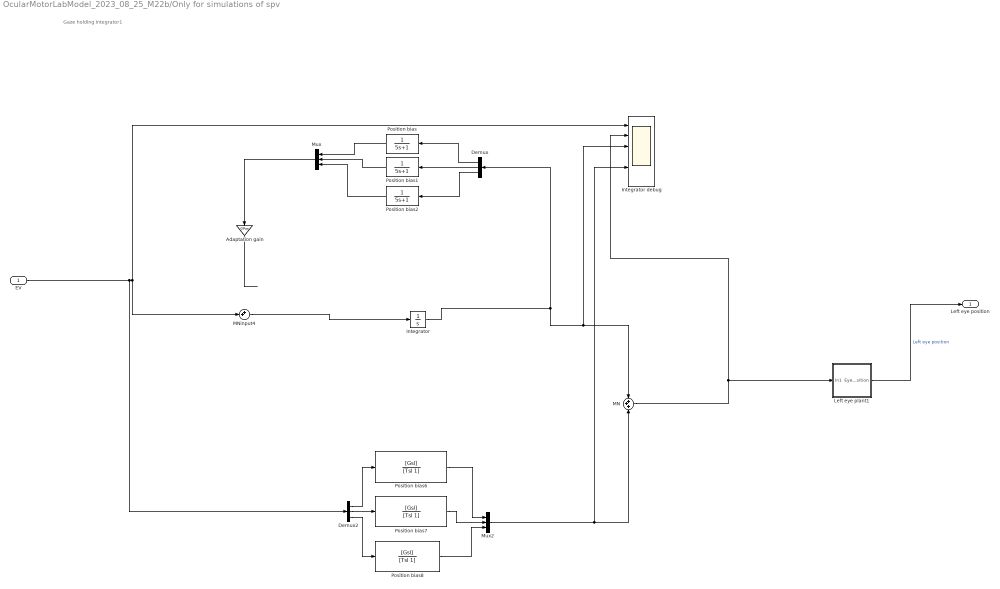
== system OcularMotorLabModel_2023_08_25_M22b/Only for simulations of spv ==
  note: Gaze holding Integrator1
  EV : Inport
  Adaptation gain : Gain  Gain=GPos
  Demux : Demux  Outputs=3
  Demux2 : Demux  Outputs=3
  Integrator : Integrator
  Integrator debug : Scope  NumInputPorts=6
  Left eye plant1 : Subsystem
  "MN " : Sum  Inputs=+++  InputSameDT=on  SaturateOnIntegerOverflow=on  OutDataTypeStr=Inherit: Same as first input
  MNinput4 : Sum  Inputs=++|  InputSameDT=on  SaturateOnIntegerOverflow=on  OutDataTypeStr=Inherit: Same as first input
  Mux : Mux  Inputs=3
  Mux2 : Mux  Inputs=3
  Position bias : TransferFcn  Numerator=1  Denominator=[5 1]
  Position bias1 : TransferFcn  Numerator=1  Denominator=[5 1]
  Position bias2 : TransferFcn  Numerator=1  Denominator=[5 1]
  Position bias6 : TransferFcn  Numerator=[Gsl]  Denominator=[Tsl 1]
  Position bias7 : TransferFcn  Numerator=[Gsl]  Denominator=[Tsl 1]
  Position bias8 : TransferFcn  Numerator=[Gsl]  Denominator=[Tsl 1]
  Left eye position : Outport
  wires:
  "MN "/1 -> Left eye plant1/1(In1), Integrator debug/2
  Left eye plant1/1(Eye position) -> Left eye position/1  "Left eye position"
  Adaptation gain/1 -> ?
  Mux2/1 -> Integrator debug/5, "MN "/3
  Demux2/2 -> Position bias7/1
  Position bias8/1 -> Mux2/3
  Demux2/3 -> Position bias8/1
  Position bias6/1 -> Mux2/1
  Demux2/1 -> Position bias6/1
  EV/1 -> MNinput4/2, Integrator debug/1, Demux2/1
  Position bias7/1 -> Mux2/2
  Integrator/1 -> Integrator debug/3, "MN "/1, Demux/1
  MNinput4/1 -> Integrator/1
  Position bias2/1 -> Mux/3
  Position bias/1 -> Mux/1
  Position bias1/1 -> Mux/2
  Demux/3 -> Position bias2/1
  Demux/2 -> Position bias1/1
  Demux/1 -> Position bias/1
  Mux/1 -> Adaptation gain/1

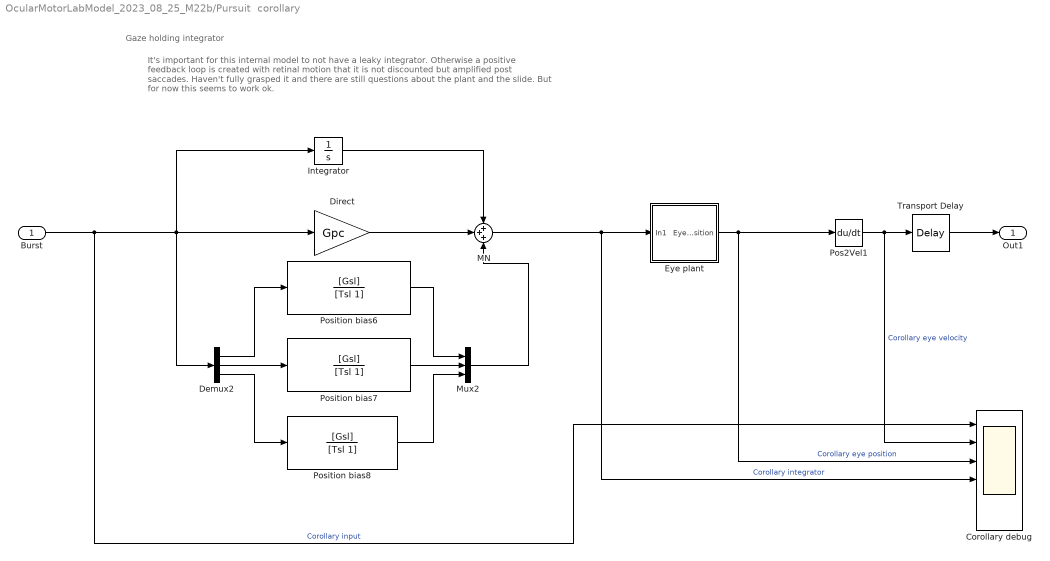
== system OcularMotorLabModel_2023_08_25_M22b/Pursuit  corollary ==
  note: Gaze holding integrator
  note: It's important for this internal model to not have a leaky integrator. Otherwise a positive feedback loop is created with retinal motion that it is not discounted but amplified post saccades.
      |
      | Haven't fully grasped it and there are still questions about the plant and the slide. But for now this seems to work ok.
  Burst : Inport
  Corollary debug : Scope  NumInputPorts=6
  Demux2 : Demux  Outputs=3
  Direct : Gain  Gain=Gpc
  Eye plant : Subsystem
  Integrator : Integrator
  "MN " : Sum  Inputs=+++  InputSameDT=on  SaturateOnIntegerOverflow=on  OutDataTypeStr=Inherit: Same as first input
  Mux2 : Mux  Inputs=3
  Pos2Vel1 : Derivative
  Position bias6 : TransferFcn  Numerator=[Gsl]  Denominator=[Tsl 1]
  Position bias7 : TransferFcn  Numerator=[Gsl]  Denominator=[Tsl 1]
  Position bias8 : TransferFcn  Numerator=[Gsl]  Denominator=[Tsl 1]
  Transport Delay : TransportDelay  DelayTime=tdv+tdm
  Out1 : Outport
  wires:
  Burst/1 -> Integrator/1, Direct/1, Demux2/1, Corollary debug/1  "Corollary input"
  Eye plant/1(Eye position) -> Pos2Vel1/1, Corollary debug/3  "Corollary eye position"
  "MN "/1 -> Eye plant/1(In1), Corollary debug/4  "Corollary integrator"
  Transport Delay/1 -> Out1/1
  Pos2Vel1/1 -> Corollary debug/2, Transport Delay/1  "Corollary eye velocity"
  Mux2/1 -> "MN "/3
  Integrator/1 -> "MN "/1
  Demux2/2 -> Position bias7/1
  Position bias8/1 -> Mux2/3
  Demux2/3 -> Position bias8/1
  Position bias6/1 -> Mux2/1
  Demux2/1 -> Position bias6/1
  Position bias7/1 -> Mux2/2
  Direct/1 -> "MN "/2

== system OcularMotorLabModel_2023_08_25_M22b/Right eye plant ==
  In1 : Inport
  Demux : Demux  Outputs=3
  Mux : Mux  Inputs=3
  Plant1 : TransferFcn  Numerator=[Tz 1]  Denominator=[T1*T2 (T1+T2) 1]
  Plant2 : TransferFcn  Numerator=[w^2]  Denominator=[1 + 2*psi*w w^2]
  Plant3 : TransferFcn  Numerator=[Tz 1]  Denominator=[T1*T2 (T1+T2) 1]
  Plant4 : TransferFcn  Numerator=[w^2]  Denominator=[1 + 2*psi*w w^2]
  Plant5 : TransferFcn  Numerator=[Tz 1]  Denominator=[T1*T2 (T1+T2) 1]
  Plant6 : TransferFcn  Numerator=[w^2]  Denominator=[1 + 2*psi*w w^2]
  Saturation : Saturate  UpperLimit=50*pi/180  LowerLimit=-50*pi/180
  Eye position : Outport
  wires:
  In1/1 -> Demux/1
  Mux/1 -> Saturation/1  "Eye position"
  Plant4/1 -> Mux/1
  Plant2/1 -> Mux/2
  Plant6/1 -> Mux/3
  Demux/1 -> Plant3/1
  Demux/2 -> Plant1/1
  Demux/3 -> Plant5/1
  Saturation/1 -> Eye position/1
  Plant3/1 -> Plant4/1
  Plant1/1 -> Plant2/1
  Plant5/1 -> Plant6/1

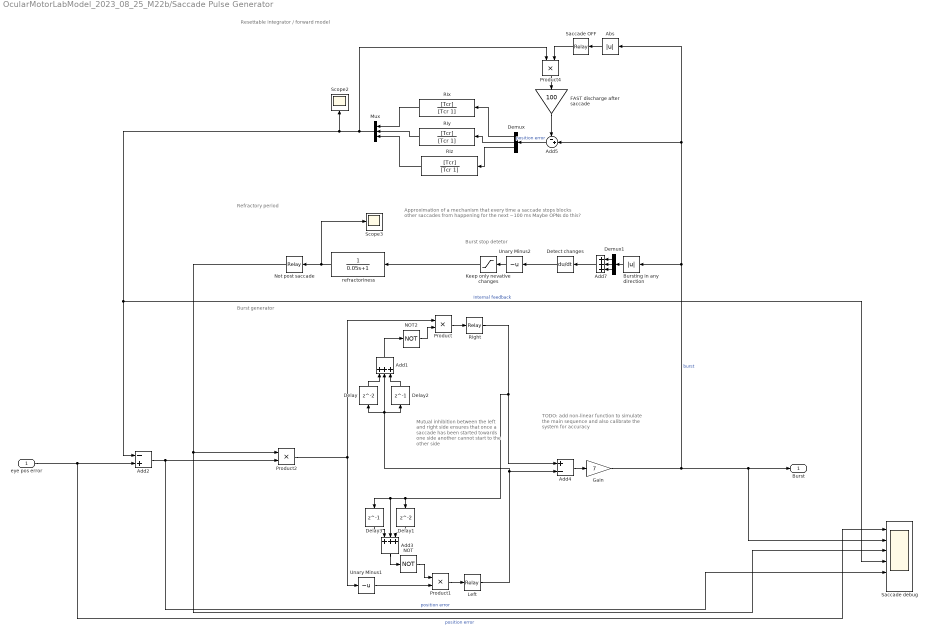
== system OcularMotorLabModel_2023_08_25_M22b/Saccade Pulse Generator ==
  note: Burst generator
  note: Resettable integrator / forward model
  note: Refractory period
  note: Burst stop detetor
  note: Mutual inhibition between the left and right side ensures that once a saccade has been started towards one side another cannot start to the other side
  note: TODO: add non-linear function to simulate the main sequence and also calibrate the system for accuracy
  note: Approximation of a mechanism that every time a saccade stops blocks other saccades from happening for the next ~100 ms
      | Maybe OPNs do this?
  eye pos error : Inport
  Abs : Abs  SaturateOnIntegerOverflow=off
  Add1 : Sum  Inputs=+++
  Add2 : Sum  Inputs=-+
  Add3 : Sum  Inputs=+++
  Add4 : Sum  Inputs=+-
  Add5 : Sum  Inputs=-+|
  Add7 : Sum  Inputs=+++
  Bursting in any direction : Abs  SaturateOnIntegerOverflow=off
  Delay : Delay  InitialCondition=0
  Delay1 : Delay  InitialCondition=0
  Delay2 : Delay  DelayLength=1  InitialCondition=0
  Delay3 : Delay  DelayLength=1  InitialCondition=0
  Demux : Demux  Outputs=3
  Demux1 : Demux  Outputs=3
  Detect changes : Derivative
  FAST discharge after saccade : Gain  Gain=100
  Gain : Gain  Gain=7
  Keep only nevative changes : Saturate  UpperLimit=50000000  LowerLimit=0
  Left : Relay  OnSwitchValue=0.2/180*pi  OffSwitchValue=0
  Mux : Mux  Inputs=3
  NOT : Logic  Operator=NOT  IconShape=distinctive  AllPortsSameDT=off  OutDataTypeStr=boolean
  NOT2 : Logic  Operator=NOT  IconShape=distinctive  AllPortsSameDT=off  OutDataTypeStr=boolean
  Not post saccade : Relay  OnSwitchValue=1  OffSwitchValue=1  OnOutputValue=0  OffOutputValue=1
  Product{,1..2,4} (4 alike) : Product
  RIx : TransferFcn  Numerator=[Tcr]  Denominator=[Tcr 1]
  RIy : TransferFcn  Numerator=[Tcr]  Denominator=[Tcr 1]
  RIz : TransferFcn  Numerator=[Tcr]  Denominator=[Tcr 1]
  Right : Relay  OnSwitchValue=0.2/180*pi  OffSwitchValue=0
  Saccade OFF : Relay  OnOutputValue=0  OffOutputValue=1
  Saccade debug : Scope  NumInputPorts=6
  Scope2 : Scope
  Scope3 : Scope
  Unary Minus1 : UnaryMinus
  Unary Minus2 : UnaryMinus
  refractoriness : TransferFcn  Numerator=1  Denominator=[0.05 1]
  Burst : Outport  VectorParamsAs1DForOutWhenUnconnected=off
  wires:
  eye pos error/1 -> Saccade debug/1, Add2/2  "position error"
  Add2/1 -> Saccade debug/5, Product2/2  "position error"
  Add7/1 -> Detect changes/1
  Detect changes/1 -> Unary Minus2/1
  Demux1/1 -> Add7/1
  Demux1/3 -> Add7/3
  Unary Minus2/1 -> Keep only nevative changes/1
  Demux1/2 -> Add7/2
  Bursting in any direction/1 -> Demux1/1
  refractoriness/1 -> Not post saccade/1, Scope3/1
  Keep only nevative changes/1 -> refractoriness/1
  Abs/1 -> Saccade OFF/1
  Product4/1 -> FAST discharge after saccade/1
  Mux/1 -> Saccade debug/4, Add2/1, Scope2/1, Product4/1  "Internal feedback"
  FAST discharge after saccade/1 -> Add5/1
  Saccade OFF/1 -> Product4/2
  Not post saccade/1 -> Saccade debug/3, Product2/1
  Add3/1 -> NOT/1
  Delay/1 -> Add1/1
  Delay2/1 -> Add1/3
  Unary Minus1/1 -> Product1/2
  Add4/1 -> Gain/1
  Product2/1 -> Product/1, Unary Minus1/1
  Add1/1 -> NOT2/1
  Product1/1 -> Left/1
  Product/1 -> Right/1
  NOT2/1 -> Product/2
  Delay1/1 -> Add3/3
  NOT/1 -> Product1/1
  Left/1 -> Add4/2, Delay2/1, Add1/2, Delay/1
  Gain/1 -> Saccade debug/2, Burst/1, Abs/1, Add5/2, Bursting in any direction/1  "burst"
  Delay3/1 -> Add3/1
  Right/1 -> Delay3/1, Add3/2, Delay1/1, Add4/1
  Demux/1 -> RIx/1
  RIy/1 -> Mux/2
  RIx/1 -> Mux/1
  Demux/3 -> RIz/1
  Demux/2 -> RIy/1
  RIz/1 -> Mux/3
  Add5/1 -> Demux/1  "position error"

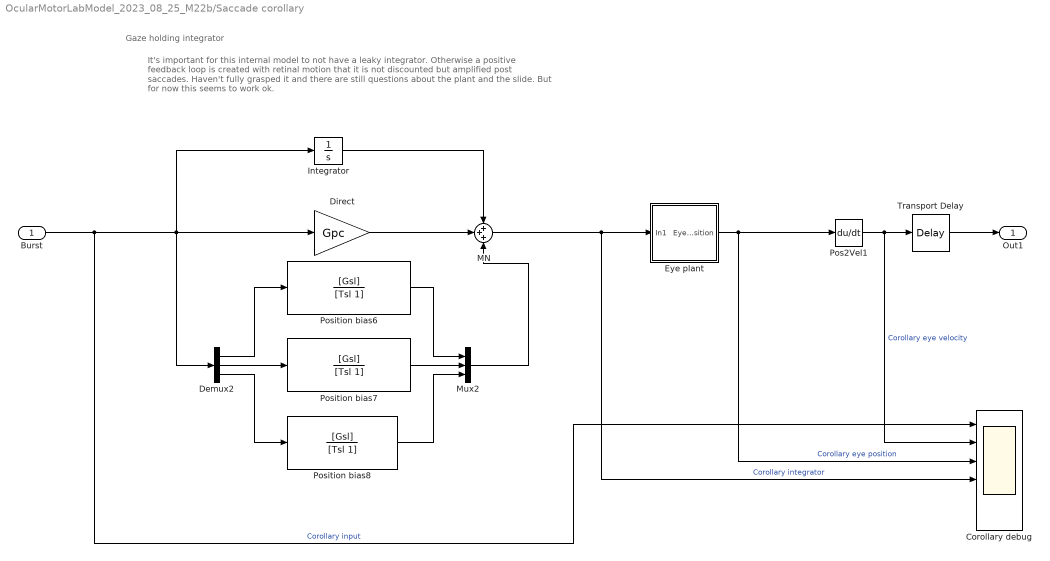
== system OcularMotorLabModel_2023_08_25_M22b/Saccade corollary ==
  note: Gaze holding integrator
  note: It's important for this internal model to not have a leaky integrator. Otherwise a positive feedback loop is created with retinal motion that it is not discounted but amplified post saccades.
      |
      | Haven't fully grasped it and there are still questions about the plant and the slide. But for now this seems to work ok.
  Burst : Inport
  Corollary debug : Scope  NumInputPorts=6
  Demux2 : Demux  Outputs=3
  Direct : Gain  Gain=Gpc
  Eye plant : Subsystem
  Integrator : Integrator
  "MN " : Sum  Inputs=+++  InputSameDT=on  SaturateOnIntegerOverflow=on  OutDataTypeStr=Inherit: Same as first input
  Mux2 : Mux  Inputs=3
  Pos2Vel1 : Derivative
  Position bias6 : TransferFcn  Numerator=[Gsl]  Denominator=[Tsl 1]
  Position bias7 : TransferFcn  Numerator=[Gsl]  Denominator=[Tsl 1]
  Position bias8 : TransferFcn  Numerator=[Gsl]  Denominator=[Tsl 1]
  Transport Delay : TransportDelay  DelayTime=tdv+tdm
  Out1 : Outport
  wires:
  Burst/1 -> Integrator/1, Direct/1, Demux2/1, Corollary debug/1  "Corollary input"
  Eye plant/1(Eye position) -> Pos2Vel1/1, Corollary debug/3  "Corollary eye position"
  "MN "/1 -> Eye plant/1(In1), Corollary debug/4  "Corollary integrator"
  Transport Delay/1 -> Out1/1
  Pos2Vel1/1 -> Corollary debug/2, Transport Delay/1  "Corollary eye velocity"
  Mux2/1 -> "MN "/3
  Integrator/1 -> "MN "/1
  Demux2/2 -> Position bias7/1
  Position bias8/1 -> Mux2/3
  Demux2/3 -> Position bias8/1
  Position bias6/1 -> Mux2/1
  Demux2/1 -> Position bias6/1
  Position bias7/1 -> Mux2/2
  Direct/1 -> "MN "/2

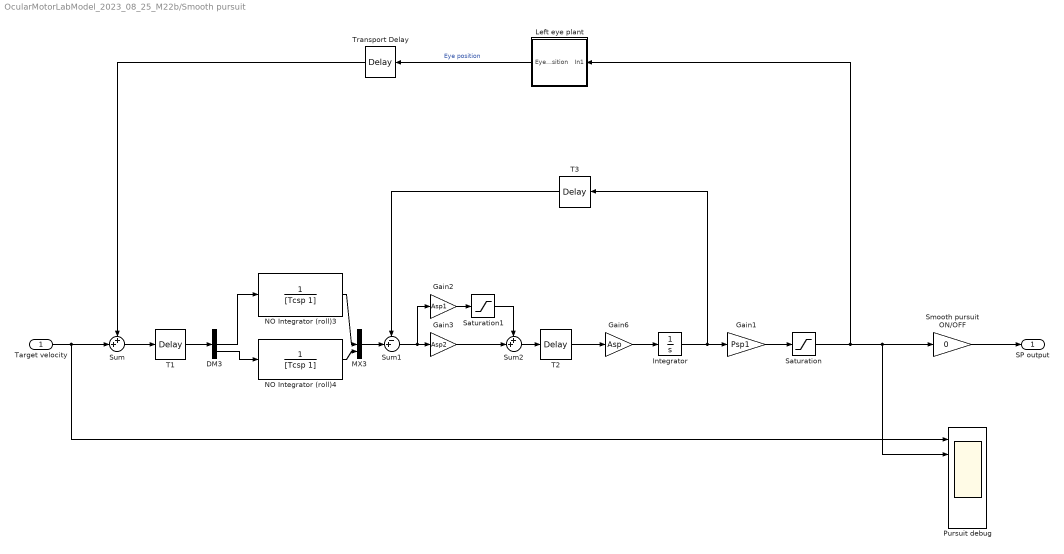
== system OcularMotorLabModel_2023_08_25_M22b/Smooth pursuit ==
  Target velocity : Inport
  DM3 : Demux  Outputs=3
  Gain1 : Gain  Gain=Psp1
  Gain2 : Gain  Gain=Asp1
  Gain3 : Gain  Gain=Asp2
  Gain6 : Gain  Gain=Asp
  Integrator : Integrator
  Left eye plant : Subsystem
  MX3 : Mux  Inputs=3
  NO Integrator (roll)3 : TransferFcn  Denominator=[Tcsp 1]
  NO Integrator (roll)4 : TransferFcn  Denominator=[Tcsp 1]
  Pursuit debug : Scope  NumInputPorts=6
  Saturation : Saturate  UpperLimit=deg2rad(SatSp)  LowerLimit=-deg2rad(SatSp)
  Saturation1 : Saturate  UpperLimit=deg2rad(e0sp)  LowerLimit=-deg2rad(e0sp)
  Smooth pursuit ON/OFF : Gain  Gain=0
  Sum : Sum  Inputs=++|
  Sum1 : Sum  Inputs=-+|
  Sum2 : Sum  Inputs=++|
  T1 : TransportDelay  DelayTime=tdsp1
  T2 : TransportDelay  DelayTime=tdsp2
  T3 : TransportDelay  DelayTime=tdsp3
  Transport Delay : TransportDelay  DelayTime=tdv+tdm
  SP output : Outport
  wires:
  Target velocity/1 -> Pursuit debug/1, Sum/2
  Sum/1 -> T1/1
  Saturation/1 -> Left eye plant/1(In1), Pursuit debug/2, Smooth pursuit ON/OFF/1
  Left eye plant/1(Eye position) -> Transport Delay/1  "Eye position"
  Transport Delay/1 -> Sum/1
  MX3/1 -> Sum1/2
  DM3/2 -> NO Integrator (roll)3/1
  NO Integrator (roll)3/1 -> MX3/2
  DM3/3 -> NO Integrator (roll)4/1
  NO Integrator (roll)4/1 -> MX3/3
  T1/1 -> DM3/1
  Gain6/1 -> Integrator/1
  Integrator/1 -> T3/1, Gain1/1
  T2/1 -> Gain6/1
  T3/1 -> Sum1/1
  Gain1/1 -> Saturation/1
  Gain2/1 -> Saturation1/1
  Gain3/1 -> Sum2/2
  Saturation1/1 -> Sum2/1
  Sum1/1 -> Gain3/1, Gain2/1
  Sum2/1 -> T2/1
  Smooth pursuit ON/OFF/1 -> SP output/1

== system OcularMotorLabModel_2023_08_25_M22b/Target position ==
  Bus Creator : BusCreator  Tag=Bus Creator  Inputs=3
  FromWs : FromWorkspace  Tag=STV FromWs  VariableName=tuvar
      SigBuilderData=|
      | common.afterFinalStr = 'Extrapolate'
      | common.sampleTime = 0
      | dataSet(1).timeRange = [0 88]
      | dataSet(1).name = 'Fixed streight ahead'
      | dataSet(2).timeRange = [0 88]
      | dataSet(2).name = 'Saccade Left and back'
      | dataSet(3).timeRange = [0 88]
      | dataSet(3).name = 'Saccade Right and back small'
      | dataSet(4).timeRange = [0 88]
      | dataSet(4).name = 'Saccade Up down and back'
      | dataSet(5).timeRange = [0 88]
      | dataSet(5).name = 'Horizontal smooth pursuit'
      | sbobj.Groups(1).Name = 'Fixed streight ahead'
      | sbobj.Groups(1).Signals(1).Name = 'tX (m)'
      | sbobj.Groups(1).Signals(1).XData = [0 88]
      | sbobj.Groups(1).Signals(1).YData = [1 1]
      | sbobj.Groups(1).Signals(2).Name = 'tY (m)'
      | sbobj.Groups(1).Signals(2).XData = [0 5 35 88]
      | sbobj.Groups(1).Signals(2).YData = [0 0 0 0]
      | sbobj.Groups(1).Signals(3).Name = 'tZ (m)'
      | sbobj.Groups(1).Signals(3).XData = [0 88]
      | sbobj.Groups(1).Signals(3).YData = [0 0]
      | sbobj.Groups(1).TimeRange = [0 88]
      | sbobj.Groups(2).Name = 'Saccade Left and back'
      | sbobj.Groups(2).Signals(1).Name = 'tX (m)'
      | sbobj.Groups(2).Signals(1).XData = [0 88]
      | sbobj.Groups(2).Signals(1).YData = [1 1]
      | sbobj.Groups(2).Signals(2).Name = 'tY (m)'
      | sbobj.Groups(2).Signals(2).XData = [0 5 5 25.1 25.1 88]
      | sbobj.Groups(2).Signals(2).YData = [0 0 0.5 0.5 0 0]
      | sbobj.Groups(2).Signals(3).Name = 'tZ (m)'
      | sbobj.Groups(2).Signals(3).XData = [0 88]
      | sbobj.Groups(2).Signals(3).YData = [0 0]
      | sbobj.Groups(2).TimeRange = [0 88]
      | sbobj.Groups(3).Name = 'Saccade Right and back small'
      | sbobj.Groups(3).Signals(1).Name = 'tX (m)'
      | sbobj.Groups(3).Signals(1).XData = [0 88]
      | sbobj.Groups(3).Signals(1).YData = [1 1]
      | sbobj.Groups(3).Signals(2).Name = 'tY (m)'
      | sbobj.Groups(3).Signals(2).XData = [0 5 5 35 35 88]
      | sbobj.Groups(3).Signals(2).YData = [0 0 0.02 0.02 0 0]
      | sbobj.Groups(3).Signals(3).Name = 'tZ (m)'
      | sbobj.Groups(3).Signals(3).XData = [0 88]
      | sbobj.Groups(3).Signals(3).YData = [0 0]
      | sbobj.Groups(3).TimeRange = [0 88]
      | sbobj.Groups(4).Name = 'Saccade Up down and back'
      | sbobj.Groups(4).Signals(1).Name = 'tX (m)'
      | sbobj.Groups(4).Signals(1).XData = [0 88]
      | sbobj.Groups(4).Signals(1).YData = [1 1]
      | sbobj.Groups(4).Signals(2).Name = 'tY (m)'
      | sbobj.Groups(4).Signals(2).XData = [0 5 35 88]
      | sbobj.Groups(4).Signals(2).YData = [0 0 0 0]
      | sbobj.Groups(4).Signals(3).Name = 'tZ (m)'
      | sbobj.Groups(4).Signals(3).XData = [0 10 10 13.1 13.1 88]
      | sbobj.Groups(4).Signals(3).YData = [0 0 0.5 0.5 0 0]
      | sbobj.Groups(4).TimeRange = [0 88]
      | sbobj.Groups(5).Name = 'Horizontal smooth pursuit'
      | sbobj.Groups(5).Signals(1).Name = 'tX (m)'
      | sbobj.Groups(5).Signals(1).XData = [0 88]
      | sbobj.Groups(5).Signals(1).YData = [1 1]
      | sbobj.Groups(5).Signals(2).Name = 'tY (m)'
      | sbobj.Groups(5).Signals(2).XData = [0 10 20 20 88]
      | sbobj.Groups(5).Signals(2).YData = [0 0 0.5 0 0]
      | sbobj.Groups(5).Signals(3).Name = 'tZ (m)'
      | sbobj.Groups(5).Signals(3).XData = [0 10 20 88]
      | sbobj.Groups(5).Signals(3).YData = [0 0 0 0]
      | sbobj.Groups(5).TimeRange = [0 88]
  Subsystem : Subsystem
  Bus : Outport
  wires:
  FromWs/1 -> Subsystem/1(In1)
  Subsystem/1(tX (m)) -> Bus Creator/1  "tX (m)"
  Subsystem/2(tY (m)) -> Bus Creator/2  "tY (m)"
  Subsystem/3(tZ (m)) -> Bus Creator/3  "tZ (m)"
  Bus Creator/1 -> Bus/1

== system OcularMotorLabModel_2023_08_25_M22b/Velocity storage ==
  In1 : Inport
  DM : Demux  Outputs=3
  IA Integrator (pitch) : TransferFcn  Numerator=1  Denominator=[TCvs 1]
  MX : Mux  Inputs=3
  NO Integrator (roll) : TransferFcn  Numerator=1  Denominator=[TCvs 1]
  RC Integrator (yaw) : TransferFcn  Numerator=1  Denominator=[TCvs 1]
  Out1 : Outport
  wires:
  MX/1 -> Out1/1
  DM/3 -> RC Integrator (yaw)/1
  RC Integrator (yaw)/1 -> MX/3
  IA Integrator (pitch)/1 -> MX/2
  NO Integrator (roll)/1 -> MX/1
  DM/1 -> NO Integrator (roll)/1
  In1/1 -> DM/1
  DM/2 -> IA Integrator (pitch)/1

== system OcularMotorLabModel_2023_08_25_M22b/Vergence ==
  In1 : Inport
  Vergence on/off : Gain
  Out1 : Outport
  wires:
  Vergence on/off/1 -> Out1/1
  In1/1 -> Vergence on/off/1

== system OcularMotorLabModel_2023_08_25_M22b/Vergence integrator ==
  In1 : Inport
  Vergence integrator : Gain
  Out1 : Outport
  wires:
  In1/1 -> Vergence integrator/1
  Vergence integrator/1 -> Out1/1

== system OcularMotorLabModel_2023_08_25_M22b/Visual World Extrinsic Orientation (only for unidirectional reotations) ==
  Bus Creator : BusCreator  Tag=Bus Creator  Inputs=3
  FromWs : FromWorkspace  Tag=STV FromWs  VariableName=tuvar
      SigBuilderData=|
      | common.afterFinalStr = 'Extrapolate'
      | common.sampleTime = 0
      | dataSet(1).timeRange = [0 60]
      | dataSet(1).name = 'Roll 0.2 Hz'
      | dataSet(2).timeRange = [0 60]
      | dataSet(2).name = 'Roll 0.1 Hz'
      | dataSet(3).timeRange = [0 60]
      | dataSet(3).name = 'Roll 0.05 Hz'
      | dataSet(4).timeRange = [0 60]
      | dataSet(4).name = 'Roll 0.2 Hz IA'
      | dataSet(5).timeRange = [0 60]
      | dataSet(5).name = 'Roll 0.1 Hz IA'
      | dataSet(6).timeRange = [0 60]
      | dataSet(6).name = 'Roll 0.05 Hz IA'
      | dataSet(7).timeRange = [0 60]
      | dataSet(7).name = 'Roll 0.2 Hz RC'
      | dataSet(8).timeRange = [0 60]
      | dataSet(8).name = 'Roll 0.1 Hz RC'
      | dataSet(9).timeRange = [0 60]
      | dataSet(9).name = 'Roll 0.05 Hz RC'
      | dataSet(10).timeRange = [0 60]
      | dataSet(10).name = 'Zeros'
      | dataSet(11).timeRange = [0 60]
      | dataSet(11).name = 'SimpleSims'
      | sbobj.Groups(1).Name = 'Roll 0.2 Hz'
      | sbobj.Groups(1).Signals(1).Name = 'N-O (roll)'
      | sbobj.Groups(1).Signals(1).XData = [0 0.00500500500501 0.01001001001 0.015015015015 0.02002002002 0.025025025025 0.03003003003 0.035035035035 0.04004004004 0.045045045045 0.0500500500501 0.0550550550551 ... (11989 elements, 1x11989)]
      | sbobj.Groups(1).Signals(1).YData = [0 0.125788666321 0.251572356775 0.377346095689 0.503104907788 0.628843818382 0.754557853574 0.880242040448 1.00589140727 1.13150098368 1.25706580089 1.3825808919 ... (11989 elements, 1x11989)]
      | sbobj.Groups(1).Signals(2).Name = 'I-A (pitch)'
      | sbobj.Groups(1).Signals(2).XData = [0 60]
      | sbobj.Groups(1).Signals(2).YData = [0 0]
      | sbobj.Groups(1).Signals(3).Name = 'R-C (yaw)'
      | sbobj.Groups(1).Signals(3).XData = [0 60]
      | sbobj.Groups(1).Signals(3).YData = [0 0]
      | sbobj.Groups(1).TimeRange = [0 60]
      | sbobj.Groups(2).Name = 'Roll 0.1 Hz'
      | sbobj.Groups(2).Signals(1).Name = 'N-O (roll)'
      | sbobj.Groups(2).Signals(1).XData = [0 0.01001001001 0.02002002002 0.03003003003 0.04004004004 0.0500500500501 0.0600600600601 0.0700700700701 0.0800800800801 0.0900900900901 0.1001001001 0.11011011011 ... (5995 elements, 1x5995)]
      | sbobj.Groups(2).Signals(1).YData = [0 0.125788666321 0.251572356775 0.377346095689 0.503104907788 0.628843818382 0.754557853574 0.880242040448 1.00589140727 1.13150098368 1.25706580089 1.3825808919 ... (5995 elements, 1x5995)]
      | sbobj.Groups(2).Signals(2).Name = 'I-A (pitch)'
      | sbobj.Groups(2).Signals(2).XData = [0 60]
      | sbobj.Groups(2).Signals(2).YData = [0 0]
      | sbobj.Groups(2).Signals(3).Name = 'R-C (yaw)'
      | sbobj.Groups(2).Signals(3).XData = [0 60]
      | sbobj.Groups(2).Signals(3).YData = [0 0]
      | sbobj.Groups(2).TimeRange = [0 60]
      | sbobj.Groups(3).Name = 'Roll 0.05 Hz'
      | sbobj.Groups(3).Signals(1).Name = 'N-O (roll)'
      | sbobj.Groups(3).Signals(1).XData = [0 0.02002002002 0.04004004004 0.0600600600601 0.0800800800801 0.1001001001 0.12012012012 0.14014014014 0.16016016016 0.18018018018 0.2002002002 0.22022022022 ... (2998 elements, 1x2998)]
      | sbobj.Groups(3).Signals(1).YData = [0 0.125788666321 0.251572356775 0.377346095689 0.503104907788 0.628843818382 0.754557853574 0.880242040448 1.00589140727 1.13150098368 1.25706580089 1.3825808919 ... (2998 elements, 1x2998)]
      | sbobj.Groups(3).Signals(2).Name = 'I-A (pitch)'
      | sbobj.Groups(3).Signals(2).XData = [0 60]
      | sbobj.Groups(3).Signals(2).YData = [0 0]
      | sbobj.Groups(3).Signals(3).Name = 'R-C (yaw)'
      | sbobj.Groups(3).Signals(3).XData = [0 60]
      | sbobj.Groups(3).Signals(3).YData = [0 0]
      | sbobj.Groups(3).TimeRange = [0 60]
      | sbobj.Groups(4).Name = 'Roll 0.2 Hz IA'
      | sbobj.Groups(4).Signals(1).Name = 'N-O (roll)'
      | sbobj.Groups(4).Signals(1).XData = [0 60]
      | sbobj.Groups(4).Signals(1).YData = [0 0]
      | sbobj.Groups(4).Signals(2).Name = 'I-A (pitch)'
      | sbobj.Groups(4).Signals(2).XData = [0 0.00500500500501 0.01001001001 0.015015015015 0.02002002002 0.025025025025 0.03003003003 0.035035035035 0.04004004004 0.045045045045 0.0500500500501 0.0550550550551 ... (11989 elements, 1x11989)]
      | sbobj.Groups(4).Signals(2).YData = [0 0.125788666321 0.251572356775 0.377346095689 0.503104907788 0.628843818382 0.754557853574 0.880242040448 1.00589140727 1.13150098368 1.25706580089 1.3825808919 ... (11989 elements, 1x11989)]
      | sbobj.Groups(4).Signals(3).Name = 'R-C (yaw)'
      | sbobj.Groups(4).Signals(3).XData = [0 60]
      | sbobj.Groups(4).Signals(3).YData = [0 0]
      | sbobj.Groups(4).TimeRange = [0 60]
      | sbobj.Groups(5).Name = 'Roll 0.1 Hz IA'
      | sbobj.Groups(5).Signals(1).Name = 'N-O (roll)'
      | sbobj.Groups(5).Signals(1).XData = [0 60]
      | sbobj.Groups(5).Signals(1).YData = [0 0]
      | sbobj.Groups(5).Signals(2).Name = 'I-A (pitch)'
      | sbobj.Groups(5).Signals(2).XData = [0 0.01001001001 0.02002002002 0.03003003003 0.04004004004 0.0500500500501 0.0600600600601 0.0700700700701 0.0800800800801 0.0900900900901 0.1001001001 0.11011011011 ... (5995 elements, 1x5995)]
      | sbobj.Groups(5).Signals(2).YData = [0 0.125788666321 0.251572356775 0.377346095689 0.503104907788 0.628843818382 0.754557853574 0.880242040448 1.00589140727 1.13150098368 1.25706580089 1.3825808919 ... (5995 elements, 1x5995)]
      | sbobj.Groups(5).Signals(3).Name = 'R-C (yaw)'
      | sbobj.Groups(5).Signals(3).XData = [0 60]
      | sbobj.Groups(5).Signals(3).YData = [0 0]
      | sbobj.Groups(5).TimeRange = [0 60]
      | sbobj.Groups(6).Name = 'Roll 0.05 Hz IA'
      | sbobj.Groups(6).Signals(1).Name = 'N-O (roll)'
      | sbobj.Groups(6).Signals(1).XData = [0 60]
      | sbobj.Groups(6).Signals(1).YData = [0 0]
      | sbobj.Groups(6).Signals(2).Name = 'I-A (pitch)'
      | sbobj.Groups(6).Signals(2).XData = [0 0.02002002002 0.04004004004 0.0600600600601 0.0800800800801 0.1001001001 0.12012012012 0.14014014014 0.16016016016 0.18018018018 0.2002002002 0.22022022022 ... (2998 elements, 1x2998)]
      | sbobj.Groups(6).Signals(2).YData = [0 0.125788666321 0.251572356775 0.377346095689 0.503104907788 0.628843818382 0.754557853574 0.880242040448 1.00589140727 1.13150098368 1.25706580089 1.3825808919 ... (2998 elements, 1x2998)]
      | sbobj.Groups(6).Signals(3).Name = 'R-C (yaw)'
      | sbobj.Groups(6).Signals(3).XData = [0 60]
      | sbobj.Groups(6).Signals(3).YData = [0 0]
      | sbobj.Groups(6).TimeRange = [0 60]
      | sbobj.Groups(7).Name = 'Roll 0.2 Hz RC'
      | sbobj.Groups(7).Signals(1).Name = 'N-O (roll)'
      | sbobj.Groups(7).Signals(1).XData = [0 60]
      | sbobj.Groups(7).Signals(1).YData = [0 0]
      | sbobj.Groups(7).Signals(2).Name = 'I-A (pitch)'
      | sbobj.Groups(7).Signals(2).XData = [0 60]
      | sbobj.Groups(7).Signals(2).YData = [0 0]
      | sbobj.Groups(7).Signals(3).Name = 'R-C (yaw)'
      | sbobj.Groups(7).Signals(3).XData = [0 0.00500500500501 0.01001001001 0.015015015015 0.02002002002 0.025025025025 0.03003003003 0.035035035035 0.04004004004 0.045045045045 0.0500500500501 0.0550550550551 ... (11989 elements, 1x11989)]
      | sbobj.Groups(7).Signals(3).YData = [0 0.125788666321 0.251572356775 0.377346095689 0.503104907788 0.628843818382 0.754557853574 0.880242040448 1.00589140727 1.13150098368 1.25706580089 1.3825808919 ... (11989 elements, 1x11989)]
      | sbobj.Groups(7).TimeRange = [0 60]
      | sbobj.Groups(8).Name = 'Roll 0.1 Hz RC'
      | sbobj.Groups(8).Signals(1).Name = 'N-O (roll)'
      | sbobj.Groups(8).Signals(1).XData = [0 60]
      | sbobj.Groups(8).Signals(1).YData = [0 0]
      | sbobj.Groups(8).Signals(2).Name = 'I-A (pitch)'
      | sbobj.Groups(8).Signals(2).XData = [0 60]
      | sbobj.Groups(8).Signals(2).YData = [0 0]
      | sbobj.Groups(8).Signals(3).Name = 'R-C (yaw)'
      | sbobj.Groups(8).Signals(3).XData = [0 0.01001001001 0.02002002002 0.03003003003 0.04004004004 0.0500500500501 0.0600600600601 0.0700700700701 0.0800800800801 0.0900900900901 0.1001001001 0.11011011011 ... (5995 elements, 1x5995)]
      | sbobj.Groups(8).Signals(3).YData = [0 0.125788666321 0.251572356775 0.377346095689 0.503104907788 0.628843818382 0.754557853574 0.880242040448 1.00589140727 1.13150098368 1.25706580089 1.3825808919 ... (5995 elements, 1x5995)]
      | sbobj.Groups(8).TimeRange = [0 60]
      | sbobj.Groups(9).Name = 'Roll 0.05 Hz RC'
      | sbobj.Groups(9).Signals(1).Name = 'N-O (roll)'
      | sbobj.Groups(9).Signals(1).XData = [0 60]
      | sbobj.Groups(9).Signals(1).YData = [0 0]
      | sbobj.Groups(9).Signals(2).Name = 'I-A (pitch)'
      | sbobj.Groups(9).Signals(2).XData = [0 60]
      | sbobj.Groups(9).Signals(2).YData = [0 0]
      | sbobj.Groups(9).Signals(3).Name = 'R-C (yaw)'
      | sbobj.Groups(9).Signals(3).XData = [0 0.02002002002 0.04004004004 0.0600600600601 0.0800800800801 0.1001001001 0.12012012012 0.14014014014 0.16016016016 0.18018018018 0.2002002002 0.22022022022 ... (2998 elements, 1x2998)]
      | sbobj.Groups(9).Signals(3).YData = [0 0.125788666321 0.251572356775 0.377346095689 0.503104907788 0.628843818382 0.754557853574 0.880242040448 1.00589140727 1.13150098368 1.25706580089 1.3825808919 ... (2998 elements, 1x2998)]
      | sbobj.Groups(9).TimeRange = [0 60]
      | sbobj.Groups(10).Name = 'Zeros'
      | sbobj.Groups(10).Signals(1).Name = 'N-O (roll)'
      | sbobj.Groups(10).Signals(1).XData = [0 60]
      | sbobj.Groups(10).Signals(1).YData = [0 0]
      | sbobj.Groups(10).Signals(2).Name = 'I-A (pitch)'
      | sbobj.Groups(10).Signals(2).XData = [0 60]
      | sbobj.Groups(10).Signals(2).YData = [0 0]
      | sbobj.Groups(10).Signals(3).Name = 'R-C (yaw)'
      | sbobj.Groups(10).Signals(3).XData = [0 60]
      | sbobj.Groups(10).Signals(3).YData = [0 0]
      | sbobj.Groups(10).TimeRange = [0 60]
      | sbobj.Groups(11).Name = 'SimpleSims'
      | sbobj.Groups(11).Signals(1).Name = 'N-O (roll)'
      | sbobj.Groups(11).Signals(1).XData = [0 0.01 0.02 0.03 0.04 0.05 0.06 0.07 0.08 0.09 0.1 0.11 ... (6001 elements, 1x6001)]
      | sbobj.Groups(11).Signals(1).YData = [0 0.0628317497176 0.125662879311 0.188492768663 0.251320797667 0.314146346236 0.376968794308 0.43978752185 0.502601908867 0.565411335405 0.628215181563 0.691012827489 ... (6001 elements, 1x6001)]
      | sbobj.Groups(11).Signals(2).Name = 'I-A (pitch)'
      | sbobj.Groups(11).Signals(2).XData = [0 5 35 60]
      | sbobj.Groups(11).Signals(2).YData = [0 0 0 0]
      | sbobj.Groups(11).Signals(3).Name = 'R-C (yaw)'
      | sbobj.Groups(11).Signals(3).XData = [0 5 35 60]
      | sbobj.Groups(11).Signals(3).YData = [0 0 0 0]
      | sbobj.Groups(11).TimeRange = [0 60]
  Subsystem : Subsystem
  Bus : Outport
  wires:
  FromWs/1 -> Subsystem/1(In1)
  Subsystem/1(N-O (roll)) -> Bus Creator/1  "N-O (roll)"
  Subsystem/2(I-A (pitch)) -> Bus Creator/2  "I-A (pitch)"
  Subsystem/3(R-C (yaw)) -> Bus Creator/3  "R-C (yaw)"
  Bus Creator/1 -> Bus/1

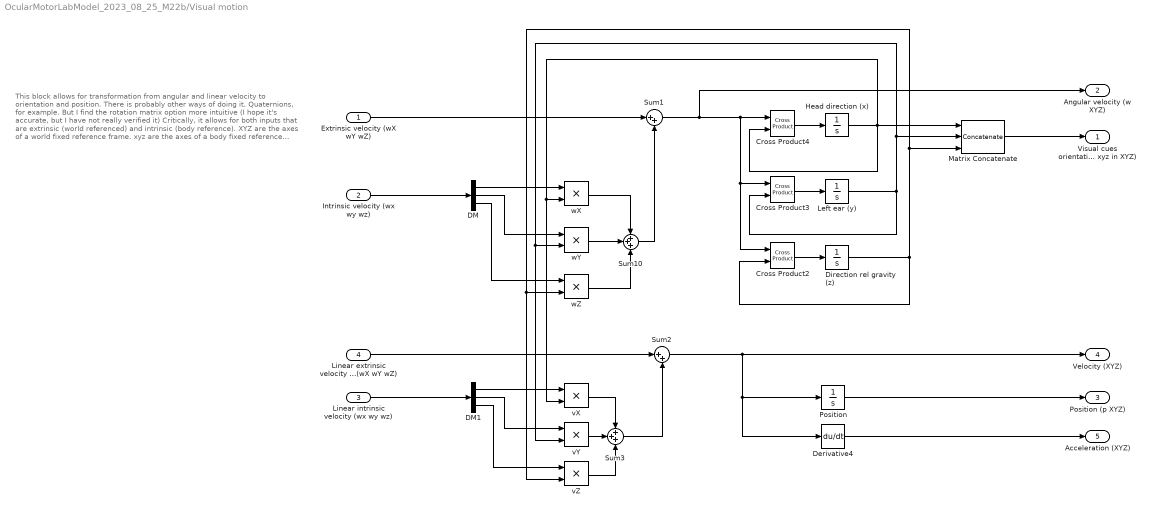
== system OcularMotorLabModel_2023_08_25_M22b/Visual motion ==
  note: This block allows for transformation from angular and linear velocity to orientation and position. There is probably other ways of doing it. Quaternions, for example. But I find the rotation matrix option more intuitive (I hope it's accurate, but I have not really verified it)
      |
      | Critically, it allows for both inputs that are extrinsic (world referenced) and intrinsic (body reference).
      |
      | XYZ are the axes of a world fixed reference frame.
      | xyz are the axes of a body fixed reference frame
      |
      | For the extrinsic angular velocities, they need to be integrated after a cross product with each of the xyz axis, that way they provide the rotation of such axis within the XYZ world fixed reference frame.
      |
      | For the intrinsic angular velocities, they simply multiply each of the intrisic axis and get added to the extrinsic velocities.
      |
      | A similar approach is followed for the linear velocities but without the cross products are linear velocities can be simply integrated by components.
  Extrinsic velocity (wX wY wZ) : Inport
  Intrinsic velocity (wx wy wz) : Inport  Port=2
  Linear intrinsic velocity (wx wy wz) : Inport  Port=3
  Linear extrinsic velocity (wX wY wZ) : Inport  Port=4
  Cross Product2 : vrlib/Utilities/Cross Product
  Cross Product3 : vrlib/Utilities/Cross Product
  Cross Product4 : vrlib/Utilities/Cross Product
  DM : Demux  Outputs=3
  DM1 : Demux  Outputs=3
  Derivative4 : Derivative
  Direction rel gravity (z) : Integrator  InitialCondition=[0 0 1]
  Head direction (x) : Integrator  InitialCondition=[1 0 0]
  Left ear (y) : Integrator  InitialCondition=[0 1 0]
  Matrix Concatenate : Concatenate  NumInputs=3  Mode=Multidimensional array  ConcatenateDimension=2
  Position : Integrator  InitialCondition=[0 0 0]
  Sum1 : Sum  Inputs=|++
  Sum10 : Sum  Inputs=+++
  Sum2 : Sum  Inputs=|++
  Sum3 : Sum  Inputs=+++
  vX : Product
  vY : Product
  vZ : Product
  wX : Product
  wY : Product
  wZ : Product
  Visual cues orientation in world (R xyz in XYZ) : Outport
  Angular velocity (w XYZ) : Outport  Port=2
  Position (p XYZ) : Outport  Port=3
  Velocity (XYZ) : Outport  Port=4
  Acceleration (XYZ) : Outport  Port=5
  wires:
  Head direction (x)/1 -> Cross Product4/2, wX/2, vX/2, Matrix Concatenate/1
  Cross Product4/1 -> Head direction (x)/1
  Direction rel gravity (z)/1 -> Matrix Concatenate/3, wZ/2, vZ/2, Cross Product2/2
  Cross Product2/1 -> Direction rel gravity (z)/1
  Left ear (y)/1 -> Matrix Concatenate/2, vY/2, wY/2, Cross Product3/2
  Sum1/1 -> Cross Product2/1, Cross Product3/1, Cross Product4/1, Angular velocity (w XYZ)/1
  Cross Product3/1 -> Left ear (y)/1
  DM/1 -> wX/1
  DM/2 -> wY/1
  DM/3 -> wZ/1
  wX/1 -> Sum10/1
  wY/1 -> Sum10/2
  wZ/1 -> Sum10/3
  Sum10/1 -> Sum1/2
  Position/1 -> Position (p XYZ)/1
  vY/1 -> Sum3/2
  DM1/2 -> vY/1
  vZ/1 -> Sum3/3
  DM1/3 -> vZ/1
  DM1/1 -> vX/1
  vX/1 -> Sum3/1
  Sum3/1 -> Sum2/2
  Matrix Concatenate/1 -> Visual cues orientation in world (R xyz in XYZ)/1
  Sum2/1 -> Position/1, Derivative4/1, Velocity (XYZ)/1
  Derivative4/1 -> Acceleration (XYZ)/1
  Intrinsic velocity (wx wy wz)/1 -> DM/1
  Linear extrinsic velocity (wX wY wZ)/1 -> Sum2/1
  Linear intrinsic velocity (wx wy wz)/1 -> DM1/1
  Extrinsic velocity (wX wY wZ)/1 -> Sum1/1
